simulink model "adaptiveCT"  (R2022a)
settings: Solver=VariableStepAuto  StartTime=0.0  StopTime=timeSpan  RelTol=1e-4
values from neighbouring files (symbols this model uses):
  B = [zeros(n);       eye(n)]    [adaptiveCT_main.m]
  K_p = 50 * eye(n)    [adaptiveCT_main.m]
  K_v = 10 * eye(n)    [adaptiveCT_main.m]
  max_tau = 100 * [1 1 1 1 1 1]    [adaptiveCT_main.m]
  P = lyap(A',Q)    [adaptiveCT_main.m]
  R = 10 * eye(n * 10)    [adaptiveCT_main.m]
undefined symbols (not defined in the file or in its folder): pi_est_0, pi_real
(part 2 of 5)

== matlab function adaptiveCT/Sistema/MATLAB Function1 ==
  data: q input; dq input; C_out output; parms input
function C_out = myCoriolis(q, dq, parms)

    % https://github.com/cdsousa/SymPyBotics

    %% Denavit-Hartenberg
    a2 = 0.4318;    a3 = 0.0203;
    d3 = 0.15005;   d4 = 0.4318;

    %% Variabili di giunto
    % q1 = q(1);  dq1 = dq(1);   ddq1 = ddq(1);
    % q2 = q(2);  dq2 = dq(2);   ddq2 = ddq(2);
    % q3 = q(3);  dq3 = dq(3);   ddq3 = ddq(3);
    % q4 = q(4);  dq4 = dq(4);   ddq4 = ddq(4);
    % q5 = q(5);  dq5 = dq(5);   ddq5 = ddq(5);
    % q6 = q(6);  dq6 = dq(6);   ddq6 = ddq(6);

    %% parms
    % (L_1xx, L_1xy, L_1xz, L_1yy, L_1yz, L_1zz, l_1x, l_1y, l_1z, m_1, L_2xx, L_2xy, L_2xz, L_2yy, L_2yz, L_2zz, l_2x, l_2y, l_2z, m_2, L_3xx, L_3xy, L_3xz, L_3yy, L_3yz, L_3zz, l_3x, l_3y, l_3z, m_3, L_4xx, L_4xy, L_4xz, L_4yy, L_4yz, L_4zz, l_4x, l_4y, l_4z, m_4, L_5xx, L_5xy, L_5xz, L_5yy, L_5yz, L_5zz, l_5x, l_5y, l_5z, m_5, L_6xx, L_6xy, L_6xz, L_6yy, L_6yz, L_6zz, l_6x, l_6y, l_6z, m_6)
    % Where:
    % L is the link inertia tensor computed about the link frame;
    % l is the link first moment of inertia;
    % m is the link mass.
    % These are the so-called barycentric parameters, with respect to which the dynamic model is linear.


    x0 = sin(q(2));
    x1 = cos(q(2));
    x2 = parms(13)*x0 + parms(15)*x1;
    x3 = ((x1)*(x1));
    x4 = -a2;
    x5 = ((x0)*(x0));
    x6 = x1*(x3*x4 + x4*x5);
    x7 = parms(19)*x6;
    x8 = x0*x7 + x1*x2;
    x9 = cos(q(3));
    x10 = x0*x9;
    x11 = sin(q(3));
    x12 = x1*x11;
    x13 = x10 + x12;
    x14 = parms(28)*x13;
    x15 = -d3;
    x16 = x12*x15;
    x17 = x10*x15 + x16;
    x18 = parms(30)*x17;
    x19 = x14 + x18;
    x20 = -x6;
    x21 = x1*x9;
    x22 = a3*((x11)*(x11)) + a3*((x9)*(x9));
    x23 = x0*x11;
    x24 = -x23;
    x25 = x20 + x21*x22 + x22*x24;
    x26 = -x17;
    x27 = x21 + x24;
    x28 = -x13;
    x29 = parms(27)*x27 + parms(29)*x28 + parms(30)*x25;
    x30 = x19*x25 + x26*x29;
    x31 = sin(q(4));
    x32 = x13*x31;
    x33 = -x32;
    x34 = d4*x33 + x25*x31;
    x35 = d3*x21;
    x36 = d3*x24 + x35;
    x37 = cos(q(4));
    x38 = x34 + x36*x37;
    x39 = -x38;
    x40 = parms(35)*x27;
    x41 = x13*x37;
    x42 = parms(33)*x41;
    x43 = parms(36)*x32 + parms(37)*x17 + x42;
    x44 = x40 + x43;
    x45 = parms(38)*x39 + x44;
    x46 = cos(q(5));
    x47 = x27*x46;
    x48 = sin(q(5));
    x49 = -x48;
    x50 = x41*x49;
    x51 = x47 + x50;
    x52 = parms(57)*x51;
    x53 = -x25;
    x54 = d4*x41 + x37*x53;
    x55 = x31*x36 + x54;
    x56 = -x55;
    x57 = cos(q(6));
    x58 = x17*x48;
    x59 = x38*x46 + x58;
    x60 = sin(q(6));
    x61 = -x60;
    x62 = x56*x57 + x59*x61;
    x63 = -parms(59);
    x64 = x27*x48;
    x65 = x41*x46;
    x66 = x64 + x65;
    x67 = x57*x66;
    x68 = x33*x60;
    x69 = x67 + x68;
    x70 = x63*x69;
    x71 = parms(60)*x62 + x52 + x70;
    x72 = x17*x46;
    x73 = x38*x49 + x72;
    x74 = -x73;
    x75 = x33*x57;
    x76 = x61*x66;
    x77 = x75 + x76;
    x78 = parms(53)*x69 + parms(55)*x77;
    x79 = parms(56)*x51;
    x80 = -parms(58);
    x81 = x56*x60 + x57*x59;
    x82 = parms(57)*x62 + x78 + x79 + x80*x81;
    x83 = -parms(57);
    x84 = parms(58)*x69 + x77*x83;
    x85 = parms(60)*x73 + x84;
    x86 = -x51;
    x87 = parms(52)*x69 + parms(54)*x77;
    x88 = parms(55)*x51;
    x89 = parms(59)*x81 + x73*x83 + x87 + x88;
    x90 = x62*x85 + x71*x74 + x77*x82 + x86*x89;
    x91 = parms(45)*x33;
    x92 = -x59;
    x93 = parms(43)*x66 + parms(46)*x51;
    x94 = parms(47)*x56 + parms(48)*x92 + x91 + x93;
    x95 = parms(48)*x66;
    x96 = -x33;
    x97 = parms(47)*x96;
    x98 = x95 + x97;
    x99 = parms(50)*x73 + x98;
    x100 = parms(53)*x51;
    x101 = parms(52)*x77;
    x102 = parms(51)*x69 + x101;
    x103 = parms(58)*x73 + x100 + x102 + x62*x63;
    x104 = parms(59)*x77;
    x105 = x51*x80;
    x106 = parms(60)*x81 + x104 + x105;
    x107 = -x69;
    x108 = x103*x51 + x106*x73 + x107*x82 - x81*x85;
    x109 = parms(44)*x33;
    x110 = parms(42)*x66 + parms(45)*x51;
    x111 = parms(47)*x74 + parms(49)*x59 + x109 + x110;
    x112 = -parms(49);
    x113 = parms(47)*x51 + x112*x66;
    x114 = parms(50)*x56 + x113;
    x115 = x108*x61 + x111*x86 + x114*x74 + x33*x94 + x56*x99 + x57*x90;
    x116 = parms(38)*x41;
    x117 = -x27;
    x118 = parms(37)*x117;
    x119 = x116 + x118;
    x120 = parms(40)*x55 + x119;
    x121 = -x77;
    x122 = x103*x121 - x106*x62 + x69*x89 + x71*x81;
    x123 = parms(42)*x33;
    x124 = parms(43)*x51;
    x125 = parms(41)*x66 + x124;
    x126 = parms(48)*x73 + x112*x56 + x123 + x125;
    x127 = parms(49)*x33;
    x128 = parms(48)*x86;
    x129 = x127 + x128;
    x130 = parms(50)*x59 + x129;
    x131 = x111*x66 + x114*x59 + x122 + x126*x96 - x130*x56;
    x132 = parms(34)*x27;
    x133 = parms(32)*x41 + parms(35)*x32;
    x134 = x132 + x133;
    x135 = parms(37)*x56 + parms(39)*x38 + x134;
    x136 = -parms(39);
    x137 = parms(37)*x32 + parms(40)*x17 + x136*x41;
    x138 = x115*x46 + x120*x17 + x131*x49 + x135*x33 + x137*x56 + x27*x45;
    x139 = -x66;
    x140 = -x108*x57 - x126*x51 - x130*x73 - x139*x94 - x60*x90 - x92*x99;
    x141 = parms(32)*x27;
    x142 = parms(31)*x41 + parms(33)*x32 + x136*x17;
    x143 = x141 + x142;
    x144 = parms(38)*x55 + x143;
    x145 = parms(39)*x27;
    x146 = parms(38)*x33;
    x147 = parms(40)*x38 + x145 + x146;
    x148 = x117*x144 + x135*x41 + x137*x38 + x140 + x147*x26;
    x149 = parms(22)*x13 + parms(25)*x27;
    x150 = parms(27)*x26 + x149;
    x151 = parms(29)*x36 + x150;
    x152 = x71*x86 + x77*x85;
    x153 = x106*x51 + x107*x85;
    x154 = x137*x41;
    x155 = x117*x147 - x130*x51 - x139*x99 - x152*x60 - x153*x57 + x154;
    x156 = d4*x37;
    x157 = x114*x86 + x152*x57 + x153*x61 + x33*x99;
    x158 = x106*x121 + x114*x66 + x130*x96 + x69*x71;
    x159 = x137*x33;
    x160 = x120*x27 + x157*x46 + x158*x49 + x159;
    x161 = d4*x31;
    x162 = x117*x151 + x138*x37 + x148*x31 + x155*x156 - x160*x161 + x30;
    x163 = -x41;
    x164 = x115*x48 + x120*x39 + x131*x46 + x144*x32 + x147*x55 + x163*x45;
    x165 = parms(28)*x117;
    x166 = parms(30)*x36 + x165;
    x167 = x13*x151 + x164 + x166*x53 + x29*x36;
    x168 = -x11;
    x169 = x117*x29;
    x170 = x155*x31 + x160*x37 + x169;
    x171 = x11*x15;
    x172 = x13*x29;
    x173 = x120*x163 + x147*x32 + x157*x48 + x158*x46 + x172;
    x174 = x173*x9;
    x175 = x19*x28;
    x176 = -x37;
    x177 = x155*x176 + x160*x31 + x166*x27 + x175;
    x178 = x177*x22;
    x179 = -x0;
    x180 = x1*x7 + x179*x2;
    x181 = -parms(19);
    x182 = x181*x3 + x181*x5;
    x183 = x0*(x15*x174 + x162*x9 + x167*x168 + x168*x178 + x170*x171 + x8) + x1*(d3*x170*x9 + x11*x162 + x167*x9 + x171*x173 + x178*x9 + x180) + x6*(-x177 + x182);
    x184 = -x1;
    x185 = parms(17)*x184 + parms(18)*x0 + parms(20)*x6;
    x186 = a2*x0;
    x187 = a2*parms(17) + parms(16) + x2;
    x188 = x11*x179 + x21;
    x189 = x179*x9;
    x190 = -x12;
    x191 = x189 + x190;
    x192 = x15*x23 + x35;
    x193 = a2*x11;
    x194 = x192 + x193;
    x195 = parms(28)*x194;
    x196 = x171*x179 - x35;
    x197 = x188*x37;
    x198 = x188*x31;
    x199 = d3*x189 + x16;
    x200 = -x186 + x189*x22 + x190*x22;
    x201 = x156*x188 + x176*x200 + x199*x31;
    x202 = a2*x9 + x22;
    x203 = x17 + x202;
    x204 = -x161;
    x205 = x204 + x54;
    x206 = x194*x31 + x205;
    x207 = -x31;
    x208 = x207 + x41;
    x209 = parms(38)*x208 + x118;
    x210 = parms(40)*x206 + x209;
    x211 = x191*x48 + x197*x46;
    x212 = -x198;
    x213 = x191*x46 + x197*x49;
    x214 = x188*x204 + x199*x37 + x200*x31;
    x215 = x196*x46 + x214*x49;
    x216 = x32 + x37;
    x217 = -x216;
    x218 = -x206;
    x219 = -parms(48);
    x220 = -x156;
    x221 = x220 + x34;
    x222 = x194*x37 + x221;
    x223 = x203*x48 + x222*x46;
    x224 = x208*x46 + x64;
    x225 = x208*x49 + x47;
    x226 = parms(43)*x224 + parms(45)*x217 + parms(46)*x225;
    x227 = parms(47)*x218 + x219*x223 + x226;
    x228 = x203*x46 + x222*x49;
    x229 = -parms(47);
    x230 = parms(48)*x224 + x217*x229;
    x231 = parms(50)*x228 + x230;
    x232 = x211*x57 + x212*x60;
    x233 = x211*x61 + x212*x57;
    x234 = x217*x57 + x224*x61;
    x235 = x218*x57 + x223*x61;
    x236 = x218*x60 + x223*x57;
    x237 = x217*x60 + x224*x57;
    x238 = parms(53)*x237 + parms(55)*x234 + parms(56)*x225;
    x239 = parms(57)*x235 + x236*x80 + x238;
    x240 = parms(58)*x237 + x234*x83;
    x241 = parms(60)*x228 + x240;
    x242 = -x201;
    x243 = x196*x48 + x214*x46;
    x244 = x242*x57 + x243*x61;
    x245 = parms(52)*x237 + parms(54)*x234 + parms(55)*x225;
    x246 = parms(59)*x236 + x228*x83 + x245;
    x247 = -x225;
    x248 = parms(57)*x225 + x237*x63;
    x249 = parms(60)*x235 + x248;
    x250 = -x228;
    x251 = parms(51)*x232 + parms(52)*x233 + parms(53)*x213 + parms(58)*x215 + x234*x239 + x235*x241 + x244*x63 + x246*x247 + x249*x250;
    x252 = parms(42)*x224 + parms(44)*x217 + parms(45)*x225;
    x253 = parms(49)*x223 + x228*x229 + x252;
    x254 = parms(47)*x225 + x112*x224;
    x255 = parms(50)*x218 + x254;
    x256 = x242*x60 + x243*x57;
    x257 = parms(51)*x237 + parms(52)*x234 + parms(53)*x225;
    x258 = parms(58)*x228 + x235*x63 + x257;
    x259 = parms(59)*x234 + x225*x80;
    x260 = parms(60)*x236 + x259;
    x261 = -x237;
    x262 = parms(52)*x232 + parms(54)*x233 + parms(55)*x213 + parms(59)*x256 + x215*x83 + x225*x258 + x228*x260 - x236*x241 + x239*x261;
    x263 = parms(41)*x211 + parms(42)*x212 + parms(43)*x213 + parms(48)*x215 + x112*x242 + x217*x227 + x218*x231 + x247*x253 + x250*x255 + x251*x57 + x262*x61;
    x264 = -x222;
    x265 = parms(33)*x208 + parms(36)*x216 + x40;
    x266 = parms(37)*x203 + parms(38)*x264 + x265;
    x267 = -parms(37);
    x268 = parms(32)*x208 + parms(35)*x216 + x132;
    x269 = parms(39)*x222 + x206*x267 + x268;
    x270 = parms(37)*x216 + x136*x208;
    x271 = parms(40)*x203 + x270;
    x272 = -x234;
    x273 = parms(53)*x232 + parms(55)*x233 + parms(56)*x213 + parms(57)*x244 - x235*x260 + x236*x249 + x237*x246 + x256*x80 + x258*x272;
    x274 = parms(41)*x224 + parms(42)*x217 + parms(43)*x225;
    x275 = parms(48)*x228 + x112*x218 + x274;
    x276 = -x217;
    x277 = parms(49)*x217 + x219*x225;
    x278 = parms(50)*x223 + x277;
    x279 = parms(43)*x211 + parms(45)*x212 + parms(46)*x213 + parms(47)*x242 - x218*x278 + x219*x243 + x223*x255 + x224*x253 + x273 + x275*x276;
    x280 = parms(31)*x197 + parms(32)*x191 + parms(33)*x198 + parms(38)*x201 + x136*x196 + x203*x210 + x217*x269 + x218*x271 + x263*x46 + x266*x27 + x279*x49;
    x281 = -x224;
    x282 = -parms(42)*x211 - parms(44)*x212 - parms(45)*x213 - parms(49)*x243 - x215*x229 + x223*x231 - x225*x275 - x227*x281 - x228*x278 - x251*x60 - x262*x57;
    x283 = -parms(38);
    x284 = parms(38)*x217 + x145;
    x285 = parms(40)*x222 + x284;
    x286 = -x203;
    x287 = parms(31)*x208 + parms(33)*x216 + x141;
    x288 = parms(38)*x206 + x136*x203 + x287;
    x289 = parms(33)*x197 + parms(35)*x191 + parms(36)*x198 + parms(37)*x196 + x117*x288 + x208*x269 + x214*x283 + x222*x271 + x282 + x285*x286;
    x290 = parms(30)*x203;
    x291 = parms(27) + x14;
    x292 = x290 + x291;
    x293 = -parms(29);
    x294 = -parms(27);
    x295 = -parms(24) + x149;
    x296 = parms(29)*x194 + x203*x294 + x295;
    x297 = parms(59)*x233 + parms(60)*x256 + x213*x80 + x234*x241 + x247*x249;
    x298 = parms(57)*x213 + parms(60)*x244 + x225*x260 + x232*x63 + x241*x261;
    x299 = parms(38)*x197 + parms(40)*x201 - parms(47)*x213 - parms(50)*x242 - x112*x211 + x117*x285 + x191*x267 + x208*x271 - x225*x278 - x231*x281 - x297*x60 - x298*x57;
    x300 = parms(49)*x212 + parms(50)*x243 + x213*x219 + x217*x231 + x247*x255 + x297*x57 + x298*x61;
    x301 = parms(48)*x211 + parms(50)*x215 + parms(58)*x232 + parms(60)*x215 + x212*x229 + x224*x255 + x233*x83 + x237*x249 + x260*x272 + x276*x278;
    x302 = parms(38)*x212 + parms(39)*x191 + parms(40)*x214 + x210*x27 + x217*x271 + x300*x46 + x301*x49;
    x303 = parms(23)*x13;
    x304 = parms(25) + parms(26)*x117 + parms(27)*x53 - x303;
    x305 = parms(21)*x188 + parms(23)*x191 + parms(28)*x196 + x117*x296 + x156*x299 + x195 + x200*x293 + x204*x302 + x25*x292 + x280*x37 + x286*x29 + x289*x31 + x304;
    x306 = parms(12)*x0;
    x307 = parms(14)*x1;
    x308 = -x208;
    x309 = parms(32)*x197 + parms(34)*x191 + parms(35)*x198 + parms(39)*x214 + x201*x267 + x206*x285 + x210*x264 + x216*x288 + x263*x48 + x266*x308 + x279*x46;
    x310 = parms(21)*x13 + parms(29)*x53;
    x311 = parms(23)*x27;
    x312 = x310 + x311;
    x313 = -parms(22);
    x314 = x312 + x313;
    x315 = parms(28)*x203 + x314;
    x316 = -parms(28);
    x317 = x165 + x293;
    x318 = parms(30)*x194 + x317;
    x319 = parms(23)*x188 + parms(26)*x191 + parms(27)*x200 + x13*x296 + x194*x29 + x199*x316 + x309 + x315 + x318*x53;
    x320 = a2*parms(20) + parms(17) + parms(19)*x179;
    x321 = -x14 + x169 + x294;
    x322 = parms(30)*x199 + x191*x316 - x290 + x299*x31 + x302*x37 + x321;
    x323 = parms(28)*x188 + parms(30)*x196 + parms(37)*x198 + parms(40)*x196 + x136*x197 + x172 + x210*x308 + x216*x285 + x300*x48 + x301*x46 + x318;
    x324 = x323*x9;
    x325 = parms(27)*x191 + parms(30)*x200 + x176*x299 + x188*x293 + x27*x318 + x28*x292 + x302*x31;
    x326 = x22*x325;
    x327 = -parms(15);
    x328 = -parms(18);
    x329 = parms(19)*x1 + x328;
    x330 = -parms(17);
    x331 = parms(12)*x1;
    x332 = parms(11)*x0 + parms(18)*x6;
    x333 = parms(13) + parms(19)*x4;
    x334 = -x183;
    x335 = parms(28)*x193;
    x336 = parms(25) + x335;
    x337 = parms(38)*x207;
    x338 = x193*x31;
    x339 = x204 + x338;
    x340 = parms(40)*x339;
    x341 = x337 + x340;
    x342 = x193*x37;
    x343 = x220 + x342;
    x344 = -x339;
    x345 = parms(32)*x207 + parms(35)*x37;
    x346 = parms(37)*x344 + parms(39)*x343 + x345;
    x347 = parms(37)*x37 + x136*x207;
    x348 = parms(40)*x202 + x347;
    x349 = x344*x348;
    x350 = x176*x346 + x202*x341 + x349;
    x351 = x202*x48 + x343*x46;
    x352 = -x351;
    x353 = parms(48)*x352;
    x354 = parms(47)*x344 + x353;
    x355 = x207*x46;
    x356 = x207*x49;
    x357 = parms(43)*x355 + parms(46)*x356;
    x358 = parms(45)*x176;
    x359 = x357 + x358;
    x360 = x354 + x359;
    x361 = x202*x46 + x343*x49;
    x362 = parms(50)*x361;
    x363 = parms(48)*x355;
    x364 = -x176;
    x365 = parms(47)*x364;
    x366 = x363 + x365;
    x367 = x362 + x366;
    x368 = -x356;
    x369 = -x361;
    x370 = parms(47)*x369 + parms(49)*x351;
    x371 = parms(42)*x355 + parms(45)*x356;
    x372 = parms(44)*x176;
    x373 = x371 + x372;
    x374 = x370 + x373;
    x375 = parms(50)*x344;
    x376 = parms(47)*x356 + x112*x355;
    x377 = x375 + x376;
    x378 = x369*x377;
    x379 = x176*x360 + x344*x367 + x368*x374 + x378;
    x380 = x176*x57;
    x381 = x355*x61;
    x382 = x380 + x381;
    x383 = x344*x57 + x351*x61;
    x384 = x344*x60 + x351*x57;
    x385 = parms(57)*x383 + x384*x80;
    x386 = x176*x60;
    x387 = x355*x57;
    x388 = x386 + x387;
    x389 = parms(53)*x388 + parms(55)*x382;
    x390 = parms(56)*x356;
    x391 = x389 + x390;
    x392 = x385 + x391;
    x393 = parms(60)*x361;
    x394 = parms(58)*x388 + x382*x83;
    x395 = x393 + x394;
    x396 = x383*x395;
    x397 = parms(59)*x384 + x361*x83;
    x398 = parms(52)*x388 + parms(54)*x382;
    x399 = parms(55)*x356;
    x400 = x398 + x399;
    x401 = x397 + x400;
    x402 = parms(60)*x383;
    x403 = parms(57)*x356;
    x404 = x388*x63;
    x405 = x403 + x404;
    x406 = x402 + x405;
    x407 = x368*x401 + x369*x406 + x382*x392 + x396;
    x408 = parms(58)*x361 + x383*x63;
    x409 = parms(52)*x382;
    x410 = parms(51)*x388 + x409;
    x411 = parms(53)*x356;
    x412 = x410 + x411;
    x413 = x408 + x412;
    x414 = parms(60)*x384;
    x415 = parms(59)*x382;
    x416 = x356*x80;
    x417 = x415 + x416;
    x418 = x414 + x417;
    x419 = -x388;
    x420 = -x384;
    x421 = x395*x420;
    x422 = x356*x413 + x361*x418 + x392*x419 + x421;
    x423 = x379 + x407*x57 + x422*x61;
    x424 = x351*x377;
    x425 = parms(48)*x361 + x112*x344;
    x426 = parms(43)*x356;
    x427 = parms(41)*x355 + x426;
    x428 = parms(42)*x176;
    x429 = x427 + x428;
    x430 = x425 + x429;
    x431 = -x344;
    x432 = parms(50)*x351;
    x433 = parms(49)*x176;
    x434 = parms(48)*x368;
    x435 = x433 + x434;
    x436 = x432 + x435;
    x437 = x355*x374 + x364*x430 + x424 + x431*x436;
    x438 = -x382;
    x439 = -x383;
    x440 = x384*x406 + x388*x401 + x413*x438 + x418*x439;
    x441 = x437 + x440;
    x442 = x350 + x423*x46 + x441*x49;
    x443 = x343*x348;
    x444 = -x202;
    x445 = parms(38)*x176;
    x446 = parms(40)*x343 + x445;
    x447 = x207*x346 + x443 + x444*x446;
    x448 = -x355;
    x449 = x352*x367 + x356*x430 + x360*x448 + x361*x436;
    x450 = -x407*x60 - x422*x57 - x449;
    x451 = x447 + x450;
    x452 = x356*x436 + x367*x448;
    x453 = x382*x395;
    x454 = x368*x406 + x453;
    x455 = x395*x419;
    x456 = x356*x418 + x455;
    x457 = x207*x348;
    x458 = -x452 - x454*x60 - x456*x57 + x457;
    x459 = x368*x377;
    x460 = x176*x367 + x459;
    x461 = x454*x57 + x456*x61 + x460;
    x462 = x176*x348;
    x463 = x355*x377;
    x464 = x364*x436 + x463;
    x465 = x388*x406 + x418*x438 + x464;
    x466 = x46*x461 + x462 + x465*x49;
    x467 = x156*x458 + x204*x466 + x31*x451 + x336 + x37*x442;
    x468 = parms(28)*x202 + x313;
    x469 = parms(31)*x207;
    x470 = parms(33)*x37 + x469;
    x471 = parms(38)*x339 + x136*x202 + x470;
    x472 = parms(37)*x202;
    x473 = -x343;
    x474 = parms(33)*x207;
    x475 = parms(36)*x37;
    x476 = x474 + x475;
    x477 = parms(38)*x473 + x472 + x476;
    x478 = -x207;
    x479 = x339*x446 + x341*x473 + x37*x471 + x477*x478;
    x480 = x423*x48 + x441*x46 + x479;
    x481 = x468 + x480;
    x482 = parms(30)*x202;
    x483 = x294 - x482;
    x484 = x31*x458 + x37*x466 + x483;
    x485 = x341*x478 + x37*x446;
    x486 = parms(30)*x193;
    x487 = x293 + x486;
    x488 = x46*x465 + x461*x48 + x485 + x487;
    x489 = x488*x9;
    x490 = x176*x458 + x31*x466;
    x491 = x22*x490;
    x492 = x0*(x15*x489 + x168*x481 + x168*x491 + x171*x484 + x327 + x467*x9) + x1*(d3*x484*x9 + x11*x467 + x171*x488 + x333 + x481*x9 + x491*x9) - x490*x6;
    x493 = -x492;
    x494 = -x192;
    x495 = x27*x37;
    x496 = x27*x31;
    x497 = a3*x28;
    x498 = x156*x27 + x17*x31 + x176*x497;
    x499 = a3 + x17;
    x500 = x192*x37;
    x501 = x221 + x500;
    x502 = parms(37)*x499 + x265 + x283*x501;
    x503 = x192*x31;
    x504 = x205 + x503;
    x505 = parms(40)*x504 + x209;
    x506 = x28*x48 + x46*x495;
    x507 = -x496;
    x508 = x28*x46 + x49*x495;
    x509 = x117*x161 + x17*x37 + x31*x497;
    x510 = x46*x494 + x49*x509;
    x511 = -x504;
    x512 = x46*x501 + x48*x499;
    x513 = parms(47)*x511 + x219*x512 + x226;
    x514 = x46*x499 + x49*x501;
    x515 = parms(50)*x514 + x230;
    x516 = x506*x57 + x507*x60;
    x517 = x506*x61 + x507*x57;
    x518 = x511*x57 + x512*x61;
    x519 = x511*x60 + x512*x57;
    x520 = parms(57)*x518 + x238 + x519*x80;
    x521 = parms(60)*x514 + x240;
    x522 = -x498;
    x523 = x46*x509 + x48*x494;
    x524 = x522*x57 + x523*x61;
    x525 = parms(59)*x519 + x245 + x514*x83;
    x526 = parms(60)*x518 + x248;
    x527 = -x514;
    x528 = parms(51)*x516 + parms(52)*x517 + parms(53)*x508 + parms(58)*x510 + x234*x520 + x247*x525 + x518*x521 + x524*x63 + x526*x527;
    x529 = parms(49)*x512 + x229*x514 + x252;
    x530 = parms(50)*x511 + x254;
    x531 = x522*x60 + x523*x57;
    x532 = parms(58)*x514 + x257 + x518*x63;
    x533 = parms(60)*x519 + x259;
    x534 = parms(52)*x516 + parms(54)*x517 + parms(55)*x508 + parms(59)*x531 + x225*x532 + x261*x520 + x510*x83 + x514*x533 - x519*x521;
    x535 = parms(41)*x506 + parms(42)*x507 + parms(43)*x508 + parms(48)*x510 + x112*x522 + x217*x513 + x247*x529 + x511*x515 + x527*x530 + x528*x57 + x534*x61;
    x536 = parms(39)*x501 + x267*x504 + x268;
    x537 = parms(40)*x499 + x270;
    x538 = parms(53)*x516 + parms(55)*x517 + parms(56)*x508 + parms(57)*x524 + x237*x525 + x272*x532 - x518*x533 + x519*x526 + x531*x80;
    x539 = parms(48)*x514 + x112*x511 + x274;
    x540 = parms(50)*x512 + x277;
    x541 = parms(43)*x506 + parms(45)*x507 + parms(46)*x508 + parms(47)*x522 + x219*x523 + x224*x529 + x276*x539 - x511*x540 + x512*x530 + x538;
    x542 = parms(31)*x495 + parms(32)*x28 + parms(33)*x496 + parms(38)*x498 + x136*x494 + x217*x536 + x27*x502 + x46*x535 + x49*x541 + x499*x505 + x511*x537;
    x543 = -parms(42)*x506 - parms(44)*x507 - parms(45)*x508 - parms(49)*x523 - x225*x539 - x229*x510 - x281*x513 + x512*x515 - x514*x540 - x528*x60 - x534*x57;
    x544 = parms(38)*x504 + x136*x499 + x287;
    x545 = parms(40)*x501 + x284;
    x546 = -x499;
    x547 = parms(33)*x495 + parms(35)*x28 + parms(36)*x496 + parms(37)*x494 + x117*x544 + x208*x536 + x283*x509 + x501*x537 + x543 + x545*x546;
    x548 = parms(30)*x499;
    x549 = x291 + x548;
    x550 = parms(29)*x192;
    x551 = x294*x499 + x295 + x550;
    x552 = parms(59)*x517 + parms(60)*x531 + x234*x521 + x247*x526 + x508*x80;
    x553 = parms(57)*x508 + parms(60)*x524 + x225*x533 + x261*x521 + x516*x63;
    x554 = parms(38)*x495 + parms(40)*x498 - parms(47)*x508 - parms(50)*x522 - x112*x506 + x117*x545 + x208*x537 - x225*x540 + x267*x28 - x281*x515 - x552*x60 - x553*x57;
    x555 = parms(49)*x507 + parms(50)*x523 + x217*x515 + x219*x508 + x247*x530 + x552*x57 + x553*x61;
    x556 = parms(48)*x506 + parms(50)*x510 + parms(58)*x516 + parms(60)*x510 + x224*x530 + x229*x507 + x237*x526 + x272*x533 + x276*x540 + x517*x83;
    x557 = parms(38)*x507 + parms(39)*x28 + parms(40)*x509 + x217*x537 + x27*x505 + x46*x555 + x49*x556;
    x558 = parms(21)*x27 + parms(23)*x28 + parms(28)*x192 + parms(28)*x494 + x117*x551 + x156*x554 + x204*x557 + x25*x549 + x29*x546 + x293*x497 + x304 + x31*x547 + x37*x542;
    x559 = parms(32)*x495 + parms(34)*x28 + parms(35)*x496 + parms(39)*x509 + x216*x544 + x267*x498 + x308*x502 + x46*x541 + x48*x535 - x501*x505 + x504*x545;
    x560 = parms(28)*x499;
    x561 = x192*x29;
    x562 = parms(30)*x192;
    x563 = x317 + x562;
    x564 = parms(26)*x28 + parms(27)*x497 + parms(28)*x26 + x13*x551 + x310 + 2*x311 + x313 + x53*x563 + x559 + x560 + x561;
    x565 = x18 + x28*x316 + x31*x554 + x321 + x37*x557 - x548;
    x566 = parms(30)*x494 + parms(37)*x496 + parms(40)*x494 + x136*x495 + x172 + x216*x545 + x293 + x308*x505 + x46*x556 + x48*x555 + x562;
    x567 = x566*x9;
    x568 = parms(27)*x28 + parms(29)*x117 + parms(30)*x497 + x176*x554 + x27*x563 + x28*x549 + x31*x557;
    x569 = x22*x568;
    x570 = parms(40)*x204;
    x571 = x337 + x570;
    x572 = -x204;
    x573 = parms(37)*x572 + parms(39)*x220 + x345;
    x574 = a3*parms(40) + x347;
    x575 = x572*x574;
    x576 = a3*x571 + x176*x573 + x575;
    x577 = a3*x48 + x220*x46;
    x578 = -x577;
    x579 = parms(48)*x578;
    x580 = parms(47)*x572 + x579;
    x581 = x359 + x580;
    x582 = a3*x46 + x220*x49;
    x583 = parms(50)*x582;
    x584 = x366 + x583;
    x585 = -x582;
    x586 = parms(47)*x585 + parms(49)*x577;
    x587 = x373 + x586;
    x588 = parms(50)*x572;
    x589 = x376 + x588;
    x590 = x585*x589;
    x591 = x176*x581 + x368*x587 + x572*x584 + x590;
    x592 = x57*x572 + x577*x61;
    x593 = x57*x577 + x572*x60;
    x594 = parms(57)*x592 + x593*x80;
    x595 = x391 + x594;
    x596 = parms(60)*x582;
    x597 = x394 + x596;
    x598 = x592*x597;
    x599 = parms(59)*x593 + x582*x83;
    x600 = x400 + x599;
    x601 = parms(60)*x592;
    x602 = x405 + x601;
    x603 = x368*x600 + x382*x595 + x585*x602 + x598;
    x604 = parms(58)*x582 + x592*x63;
    x605 = x412 + x604;
    x606 = parms(60)*x593;
    x607 = x417 + x606;
    x608 = -x593;
    x609 = x597*x608;
    x610 = x356*x605 + x419*x595 + x582*x607 + x609;
    x611 = x57*x603 + x591 + x61*x610;
    x612 = x577*x589;
    x613 = parms(48)*x582 + x112*x572;
    x614 = x429 + x613;
    x615 = -x572;
    x616 = parms(50)*x577;
    x617 = x435 + x616;
    x618 = x355*x587 + x364*x614 + x612 + x615*x617;
    x619 = -x592;
    x620 = x388*x600 + x438*x605 + x593*x602 + x607*x619;
    x621 = x618 + x620;
    x622 = x46*x611 + x49*x621 + x576;
    x623 = x220*x574;
    x624 = parms(40)*x220 + x445;
    x625 = -a3;
    x626 = x207*x573 + x623 + x624*x625;
    x627 = x356*x614 + x448*x581 + x578*x584 + x582*x617;
    x628 = -x57*x610 - x60*x603 - x627;
    x629 = x626 + x628;
    x630 = x356*x617 + x448*x584;
    x631 = x382*x597;
    x632 = x368*x602 + x631;
    x633 = x419*x597;
    x634 = x356*x607 + x633;
    x635 = x207*x574;
    x636 = -x57*x634 - x60*x632 - x630 + x635;
    x637 = x368*x589;
    x638 = x176*x584 + x637;
    x639 = x57*x632 + x61*x634 + x638;
    x640 = x176*x574;
    x641 = x355*x589;
    x642 = x364*x617 + x641;
    x643 = x388*x602 + x438*x607 + x642;
    x644 = x46*x639 + x49*x643 + x640;
    x645 = parms(25) + x156*x636 + x204*x644 + x31*x629 + x37*x622;
    x646 = a3*parms(28) + x313;
    x647 = a3*x136 + parms(38)*x204 + x470;
    x648 = a3*parms(37);
    x649 = -x220;
    x650 = parms(38)*x649 + x476 + x648;
    x651 = x204*x624 + x37*x647 + x478*x650 + x571*x649;
    x652 = x46*x621 + x48*x611 + x651;
    x653 = x646 + x652;
    x654 = parms(30)*x625 + x294;
    x655 = x31*x636 + x37*x644 + x654;
    x656 = x37*x624 + x478*x571;
    x657 = x293 + x46*x643 + x48*x639 + x656;
    x658 = x657*x9;
    x659 = x176*x636 + x31*x644;
    x660 = x22*x659;
    x661 = x0*(x15*x658 + x168*x653 + x168*x660 + x171*x655 + x645*x9) + x1*(d3*x655*x9 + x11*x645 + x171*x657 + x653*x9 + x660*x9) - x6*x659;
    x662 = -x661;
    x663 = -x193;
    x664 = x202 + x625;
    x665 = x31*x664;
    x666 = a3 + x202;
    x667 = -2*x31;
    x668 = -2*x161 + x338;
    x669 = parms(38)*x667 + parms(40)*x668;
    x670 = x37*x664;
    x671 = x46*x663 + x49*x670;
    x672 = 2*x37;
    x673 = -x672;
    x674 = x46*x667;
    x675 = x49*x667;
    x676 = -x668;
    x677 = -2*x156 + x342;
    x678 = x46*x677 + x48*x666;
    x679 = parms(43)*x674 + parms(45)*x673 + parms(46)*x675 + parms(47)*x676 + x219*x678;
    x680 = x46*x666 + x49*x677;
    x681 = parms(48)*x674 + parms(50)*x680 + x229*x673;
    x682 = x57*x673 + x61*x674;
    x683 = x57*x674 + x60*x673;
    x684 = x57*x676 + x61*x678;
    x685 = x57*x678 + x60*x676;
    x686 = parms(53)*x683 + parms(55)*x682 + parms(56)*x675 + parms(57)*x684 + x685*x80;
    x687 = parms(58)*x683 + parms(60)*x680 + x682*x83;
    x688 = -x665;
    x689 = x46*x670 + x48*x663;
    x690 = x57*x688 + x61*x689;
    x691 = parms(52)*x683 + parms(54)*x682 + parms(55)*x675 + parms(59)*x685 + x680*x83;
    x692 = -x675;
    x693 = parms(57)*x675 + parms(60)*x684 + x63*x683;
    x694 = -x680;
    x695 = parms(58)*x671 + x63*x690 + x682*x686 + x684*x687 + x691*x692 + x693*x694;
    x696 = parms(42)*x674 + parms(44)*x673 + parms(45)*x675 + parms(49)*x678 + x229*x680;
    x697 = parms(47)*x675 + parms(50)*x676 + x112*x674;
    x698 = x57*x689 + x60*x688;
    x699 = parms(51)*x683 + parms(52)*x682 + parms(53)*x675 + parms(58)*x680 + x63*x684;
    x700 = parms(59)*x682 + parms(60)*x685 + x675*x80;
    x701 = -x683;
    x702 = parms(59)*x698 + x671*x83 + x675*x699 + x680*x700 - x685*x687 + x686*x701;
    x703 = parms(48)*x671 + x112*x688 + x57*x695 + x61*x702 + x673*x679 + x676*x681 + x692*x696 + x694*x697;
    x704 = parms(32)*x667 + parms(35)*x672 + parms(39)*x677 + x267*x668;
    x705 = parms(37)*x672 + parms(40)*x666 + x136*x667;
    x706 = -x682;
    x707 = parms(57)*x690 + x683*x691 - x684*x700 + x685*x693 + x698*x80 + x699*x706;
    x708 = parms(41)*x674 + parms(42)*x673 + parms(43)*x675 + parms(48)*x680 + x112*x676;
    x709 = -x673;
    x710 = parms(49)*x673 + parms(50)*x678 + x219*x675;
    x711 = parms(47)*x688 + x219*x689 + x674*x696 - x676*x710 + x678*x697 + x707 + x708*x709;
    x712 = parms(38)*x665 + x136*x663 + x46*x703 + x49*x711 + x666*x669 + x673*x704 + x676*x705;
    x713 = -x674;
    x714 = -parms(49)*x689 - x229*x671 - x57*x702 - x60*x695 - x675*x708 + x678*x681 - x679*x713 - x680*x710;
    x715 = parms(40)*x677 + x283*x672;
    x716 = parms(37)*x663 + x283*x670 - x666*x715 + x667*x704 + x677*x705 + x714;
    x717 = parms(60)*x698 + x682*x687 + x692*x693;
    x718 = parms(60)*x690 + x675*x700 + x687*x701;
    x719 = parms(40)*x665 - parms(50)*x688 - x57*x718 - x60*x717 + x667*x705 - x675*x710 - x681*x713;
    x720 = parms(50)*x689 + x57*x717 + x61*x718 + x673*x681 + x692*x697;
    x721 = parms(50)*x671 + parms(60)*x671 + x674*x697 + x683*x693 + x700*x706 + x709*x710;
    x722 = parms(40)*x670 + x46*x720 + x49*x721 + x673*x705;
    x723 = 4*parms(25) + parms(28)*x663 + x156*x719 + x204*x722 + x31*x716 + 2*x335 + x37*x712;
    x724 = -x667;
    x725 = parms(39)*x670 + x267*x665 + x46*x711 + x48*x703 + x668*x715 - x669*x677 + x672*(parms(31)*x667 + parms(33)*x672 + parms(38)*x668 + x136*x666) + x724*(parms(33)*x667 + parms(36)*x672 + parms(37)*x666 + x283*x677);
    x726 = -4*parms(22) + 2*parms(28)*x666 + x316*x664 + x725;
    x727 = parms(30)*x666;
    x728 = -4*parms(27) + parms(30)*x664 + x31*x719 + x37*x722 - 2*x727;
    x729 = -4*parms(29) + parms(30)*x663 + parms(40)*x663 + x46*x721 + x48*x720 + 2*x486 + x669*x724 + x672*x715;
    x730 = x729*x9;
    x731 = x176*x719 + x31*x722;
    x732 = x22*x731;
    x733 = x34 + x500;
    x734 = x27 + 1;
    x735 = x283*x733;
    x736 = x43 + x735;
    x737 = parms(35)*x734 + x736;
    x738 = x33*x46;
    x739 = x33*x49;
    x740 = x503 + x54;
    x741 = -x740;
    x742 = x49*x741;
    x743 = x48*x734 + x65;
    x744 = x49*x733 + x72;
    x745 = parms(50)*x744;
    x746 = parms(48)*x743 + x745 + x97;
    x747 = x163*x60 + x57*x738;
    x748 = x163*x57 + x61*x738;
    x749 = x61*x743 + x75;
    x750 = x57*x743 + x68;
    x751 = x46*x734 + x50;
    x752 = x46*x733 + x58;
    x753 = x57*x741 + x61*x752;
    x754 = x57*x752 + x60*x741;
    x755 = parms(57)*x753 + x754*x80;
    x756 = parms(53)*x750 + parms(55)*x749 + parms(56)*x751 + x755;
    x757 = parms(60)*x744;
    x758 = parms(58)*x750 + x749*x83 + x757;
    x759 = -x733;
    x760 = x46*x741;
    x761 = x57*x759 + x61*x760;
    x762 = parms(59)*x754 + x744*x83;
    x763 = parms(52)*x750 + parms(54)*x749 + parms(55)*x751 + x762;
    x764 = -x751;
    x765 = parms(60)*x753;
    x766 = parms(57)*x751 + x63*x750 + x765;
    x767 = -x744;
    x768 = parms(51)*x747 + parms(52)*x748 + parms(53)*x739 + parms(58)*x742 + x63*x761 + x749*x756 + x753*x758 + x763*x764 + x766*x767;
    x769 = parms(47)*x741 + x219*x752;
    x770 = parms(43)*x743 + parms(46)*x751 + x769 + x91;
    x771 = parms(49)*x752 + x229*x744;
    x772 = parms(42)*x743 + parms(45)*x751 + x109 + x771;
    x773 = parms(50)*x741;
    x774 = parms(47)*x751 + x112*x743 + x773;
    x775 = x57*x760 + x60*x759;
    x776 = parms(58)*x744 + x63*x753;
    x777 = parms(51)*x750 + parms(52)*x749 + parms(53)*x751 + x776;
    x778 = parms(60)*x754;
    x779 = parms(59)*x749 + x751*x80 + x778;
    x780 = -x750;
    x781 = -x754;
    x782 = parms(52)*x747 + parms(54)*x748 + parms(55)*x739 + parms(59)*x775 + x742*x83 + x744*x779 + x751*x777 + x756*x780 + x758*x781;
    x783 = parms(41)*x738 + parms(42)*x163 + parms(43)*x739 + parms(48)*x742 + x112*x759 + x33*x770 + x57*x768 + x61*x782 + x741*x746 + x764*x772 + x767*x774;
    x784 = parms(40)*x740;
    x785 = x116 + x267*x734 + x784;
    x786 = x137*x741;
    x787 = -x749;
    x788 = -x753;
    x789 = parms(53)*x747 + parms(55)*x748 + parms(56)*x739 + parms(57)*x761 + x750*x763 + x754*x766 + x775*x80 + x777*x787 + x779*x788;
    x790 = parms(50)*x752;
    x791 = x127 + x219*x751 + x790;
    x792 = -x741;
    x793 = parms(48)*x744 + x112*x741;
    x794 = parms(41)*x743 + parms(43)*x751 + x123 + x793;
    x795 = parms(43)*x738 + parms(45)*x163 + parms(46)*x739 + parms(47)*x759 + x219*x760 + x743*x772 + x752*x774 + x789 + x791*x792 + x794*x96;
    x796 = parms(39)*x733 + x267*x740;
    x797 = parms(34)*x734 + x133 + x796;
    x798 = parms(31)*x33 + parms(38)*x733 + x17*x785 + x33*x797 + x42 + x46*x783 + x49*x795 + x734*x737 + x786;
    x799 = -x743;
    x800 = -x752;
    x801 = -parms(42)*x738 - parms(44)*x163 - parms(45)*x739 - parms(49)*x760 - x229*x742 - x57*x782 - x60*x768 - x744*x791 - x746*x800 - x751*x794 - x770*x799;
    x802 = x137*x733;
    x803 = parms(38)*x740;
    x804 = x142 + x803;
    x805 = parms(32)*x734 + x804;
    x806 = -x734;
    x807 = parms(40)*x733 + x146;
    x808 = parms(39)*x734 + x807;
    x809 = parms(33)*x33 + parms(36)*x41 + x26*x808 + x283*x741 + x41*x797 + x801 + x802 + x805*x806;
    x810 = parms(59)*x748 + parms(60)*x775 + x739*x80 + x749*x758 + x764*x766;
    x811 = parms(57)*x739 + parms(60)*x761 + x63*x747 + x751*x779 + x758*x780;
    x812 = -parms(47)*x739 - parms(50)*x759 - x112*x738 + x154 - x57*x811 - x60*x810 - x746*x799 - x751*x791 + x806*x808 + x807;
    x813 = parms(49)*x163 + parms(50)*x760 + x219*x739 + x33*x746 + x57*x810 + x61*x811 + x764*x774;
    x814 = parms(48)*x738 + parms(50)*x742 + parms(58)*x747 + parms(60)*x742 + x163*x229 + x743*x774 + x748*x83 + x750*x766 + x779*x787 + x791*x96;
    x815 = parms(40)*x741 - x116 + x159 + x46*x813 + x49*x814 + x734*x785;
    x816 = x150 + x550;
    x817 = x117*x816 + x30;
    x818 = x156*x812 + x204*x815 + x31*x809 + x37*x798 + x817;
    x819 = parms(32)*x33 + parms(35)*x41 + parms(39)*x741 + x163*x737 + x267*x733 + x32*x805 + x46*x795 + x48*x783 + x740*x808 + x759*x785;
    x820 = x165 + x562;
    x821 = x13*x816 + x53*x820 + x561;
    x822 = x819 + x821;
    x823 = x169 + x31*x812 + x37*x815;
    x824 = parms(37)*x41 + parms(39)*x96 + x163*x785 + x172 + x32*x808 + x46*x814 + x48*x813;
    x825 = x824*x9;
    x826 = x175 + x27*x820;
    x827 = x176*x812 + x31*x815 + x826;
    x828 = x22*x827;
    x829 = x49*x60;
    x830 = x48*x57;
    x831 = parms(53)*x830 + parms(55)*x829;
    x832 = parms(56)*x46;
    x833 = x831 + x832;
    x834 = parms(52)*x830 + parms(54)*x829;
    x835 = parms(55)*x46;
    x836 = x834 + x835;
    x837 = -x46;
    x838 = x829*x833 + x836*x837;
    x839 = parms(42)*x48 + parms(45)*x46;
    x840 = x837*x839;
    x841 = parms(52)*x829;
    x842 = parms(51)*x830 + x841;
    x843 = parms(53)*x46;
    x844 = x842 + x843;
    x845 = -x830;
    x846 = x46*x844 + x833*x845;
    x847 = x57*x838 + x61*x846 + x840;
    x848 = x48*x839;
    x849 = -x829;
    x850 = x830*x836 + x844*x849;
    x851 = x848 + x850;
    x852 = parms(35) + x46*x847 + x49*x851;
    x853 = parms(43)*x48 + parms(46)*x46;
    x854 = parms(41)*x48;
    x855 = parms(43)*x46;
    x856 = x854 + x855;
    x857 = x46*x856 + x49*x853;
    x858 = -x57*x846 - x60*x838 - x857;
    x859 = -parms(32);
    x860 = x858 + x859;
    x861 = parms(58)*x830 + x829*x83;
    x862 = x829*x861;
    x863 = parms(57)*x46;
    x864 = x63*x830;
    x865 = x863 + x864;
    x866 = x837*x865 + x862;
    x867 = parms(59)*x829;
    x868 = x46*x80;
    x869 = x867 + x868;
    x870 = x845*x861;
    x871 = x46*x869 + x870;
    x872 = x219*((x46)*(x46)) + x219*((x48)*(x48));
    x873 = x136 - x57*x871 - x60*x866 - x872;
    x874 = parms(47)*x46 + parms(49)*x49;
    x875 = x837*x874;
    x876 = x57*x866 + x61*x871 + x875;
    x877 = x48*x874;
    x878 = x830*x865 + x849*x869 + x877;
    x879 = x267 + x46*x876 + x49*x878;
    x880 = x156*x873 + x204*x879 + x31*x860 + x37*x852;
    x881 = x46*x851 + x48*x847;
    x882 = x46*x878 + x48*x876;
    x883 = x882*x9;
    x884 = x31*x873 + x37*x879;
    x885 = x176*x873 + x31*x879;
    x886 = x22*x885;
    x887 = x0*(x15*x883 + x168*x881 + x168*x886 + x171*x884 + x880*x9) + x1*(d3*x884*x9 + x11*x880 + x171*x882 + x881*x9 + x886*x9) - x6*x885;
    x888 = -x887;
    x889 = x344*x49;
    x890 = x355 + x48;
    x891 = x356 + x46;
    x892 = parms(43)*x890 + parms(46)*x891 + x358;
    x893 = x354 + x892;
    x894 = x380 + x61*x890;
    x895 = x386 + x57*x890;
    x896 = parms(53)*x895 + parms(55)*x894 + parms(56)*x891;
    x897 = x385 + x896;
    x898 = parms(58)*x895 + x83*x894;
    x899 = x393 + x898;
    x900 = x344*x46;
    x901 = x473*x57 + x61*x900;
    x902 = parms(52)*x895 + parms(54)*x894 + parms(55)*x891;
    x903 = x397 + x902;
    x904 = -x891;
    x905 = parms(57)*x891 + x63*x895;
    x906 = x402 + x905;
    x907 = x176*x46;
    x908 = x478*x60 + x57*x907;
    x909 = x478*x57 + x61*x907;
    x910 = x176*x49;
    x911 = parms(51)*x908 + parms(52)*x909 + parms(53)*x910;
    x912 = parms(58)*x889 + x369*x906 + x383*x899 + x63*x901 + x894*x897 + x903*x904 + x911;
    x913 = parms(48)*x890 + x365;
    x914 = x362 + x913;
    x915 = parms(42)*x890 + parms(45)*x891 + x372;
    x916 = x370 + x915;
    x917 = x473*x60 + x57*x900;
    x918 = parms(51)*x895 + parms(52)*x894 + parms(53)*x891;
    x919 = x408 + x918;
    x920 = parms(59)*x894 + x80*x891;
    x921 = x414 + x920;
    x922 = -x895;
    x923 = parms(52)*x908 + parms(54)*x909 + parms(55)*x910;
    x924 = parms(59)*x917 + x361*x921 + x420*x899 + x83*x889 + x891*x919 + x897*x922 + x923;
    x925 = parms(47)*x891 + x112*x890;
    x926 = x375 + x925;
    x927 = parms(41)*x907 + parms(42)*x478 + parms(43)*x910;
    x928 = parms(48)*x889 + x112*x473 + x176*x893 + x344*x914 + x369*x926 + x57*x912 + x61*x924 + x904*x916 + x927;
    x929 = x267 + x341;
    x930 = -x894;
    x931 = parms(53)*x908 + parms(55)*x909 + parms(56)*x910;
    x932 = parms(57)*x901 + x384*x906 + x439*x921 + x80*x917 + x895*x903 + x919*x930 + x931;
    x933 = parms(41)*x890 + parms(43)*x891 + x428;
    x934 = x425 + x933;
    x935 = x219*x891 + x433;
    x936 = x432 + x935;
    x937 = parms(43)*x907 + parms(45)*x478 + parms(46)*x910;
    x938 = parms(47)*x473 + x219*x900 + x351*x926 + x364*x934 + x431*x936 + x890*x916 + x932 + x937;
    x939 = parms(34) + x346;
    x940 = parms(31)*x176 + parms(35) + 2*x474 + x475;
    x941 = x176*x939 + x202*x929 + x349 + x46*x928 + x472 + x49*x938 + x940;
    x942 = -x890;
    x943 = parms(42)*x907 + parms(44)*x478 + parms(45)*x910;
    x944 = -parms(49)*x900 - x229*x889 - x352*x914 - x361*x936 - x57*x924 - x60*x912 - x891*x934 - x893*x942 - x943;
    x945 = parms(39) + x446;
    x946 = 2*parms(33)*x176 + parms(36)*x207 - x469 + x859;
    x947 = parms(38)*x344 + parms(39)*x202 + x207*x939 + x283*x344 + x443 + x444*x945 + x944 + x946;
    x948 = parms(59)*x909 + x80*x910;
    x949 = parms(60)*x917 + x894*x899 + x904*x906 + x948;
    x950 = parms(57)*x910 + x63*x908;
    x951 = parms(60)*x901 + x891*x921 + x899*x922 + x950;
    x952 = parms(47)*x910 + x112*x907;
    x953 = parms(38)*x37 + x136 + x445;
    x954 = -parms(50)*x473 + x457 - x57*x951 - x60*x949 - x891*x936 - x914*x942 - x952 + x953;
    x955 = parms(49)*x478 + x219*x910;
    x956 = parms(50)*x900 + x176*x914 + x57*x949 + x61*x951 + x904*x926 + x955;
    x957 = parms(58)*x908 + x83*x909;
    x958 = parms(48)*x907 + x229*x478;
    x959 = parms(50)*x889 + parms(60)*x889 + x364*x936 + x890*x926 + x895*x906 + x921*x930 + x957 + x958;
    x960 = parms(40)*x344 + x267 + x340 + x46*x956 + x462 + x49*x959;
    x961 = x156*x954 + x204*x960 + x31*x947 + x336 + x37*x941;
    x962 = parms(32)*x176 + parms(35)*x207;
    x963 = parms(37)*x473 + parms(39)*x344 + x339*x945 + x37*(parms(32) + x471) + x46*x938 + x473*x929 + x478*(parms(35) + x477) + x48*x928 + x962;
    x964 = x468 + x963;
    x965 = x31*x954 + x37*x960 + x483;
    x966 = parms(37)*x207 + x136*x176;
    x967 = x37*x945 + x46*x959 + x478*x929 + x48*x956 + x487 + x966;
    x968 = x9*x967;
    x969 = x176*x954 + x31*x960;
    x970 = x22*x969;
    x971 = x267 + x571;
    x972 = x49*x572;
    x973 = x580 + x892;
    x974 = x594 + x896;
    x975 = x596 + x898;
    x976 = x46*x572;
    x977 = x57*x649 + x61*x976;
    x978 = x599 + x902;
    x979 = x601 + x905;
    x980 = parms(58)*x972 + x585*x979 + x592*x975 + x63*x977 + x894*x974 + x904*x978 + x911;
    x981 = x583 + x913;
    x982 = x586 + x915;
    x983 = x57*x976 + x60*x649;
    x984 = x604 + x918;
    x985 = x606 + x920;
    x986 = parms(59)*x983 + x582*x985 + x608*x975 + x83*x972 + x891*x984 + x922*x974 + x923;
    x987 = x588 + x925;
    x988 = parms(48)*x972 + x112*x649 + x176*x973 + x57*x980 + x572*x981 + x585*x987 + x61*x986 + x904*x982 + x927;
    x989 = parms(34) + x573;
    x990 = parms(57)*x977 + x593*x979 + x619*x985 + x80*x983 + x895*x978 + x930*x984 + x931;
    x991 = x613 + x933;
    x992 = x616 + x935;
    x993 = parms(47)*x649 + x219*x976 + x364*x991 + x577*x987 + x615*x992 + x890*x982 + x937 + x990;
    x994 = a3*x971 + x176*x989 + x46*x988 + x49*x993 + x575 + x648 + x940;
    x995 = -parms(49)*x976 - x229*x972 - x57*x986 - x578*x981 - x582*x992 - x60*x980 - x891*x991 - x942*x973 - x943;
    x996 = parms(39) + x624;
    x997 = a3*parms(39) + parms(38)*x572 + x207*x989 + x283*x572 + x623 + x625*x996 + x946 + x995;
    x998 = parms(60)*x983 + x894*x975 + x904*x979 + x948;
    x999 = parms(60)*x977 + x891*x985 + x922*x975 + x950;
    x1000 = -parms(50)*x649 - x57*x999 - x60*x998 + x635 - x891*x992 - x942*x981 - x952 + x953;
    x1001 = parms(50)*x976 + x176*x981 + x57*x998 + x61*x999 + x904*x987 + x955;
    x1002 = parms(50)*x972 + parms(60)*x972 + x364*x992 + x890*x987 + x895*x979 + x930*x985 + x957 + x958;
    x1003 = parms(40)*x572 + x1001*x46 + x1002*x49 + x267 + x570 + x640;
    x1004 = parms(25) + x1000*x156 + x1003*x204 + x31*x997 + x37*x994;
    x1005 = parms(37)*x649 + parms(39)*x572 + x204*x996 + x37*(parms(32) + x647) + x46*x993 + x478*(parms(35) + x650) + x48*x988 + x649*x971 + x962;
    x1006 = x1005 + x646;
    x1007 = x1000*x31 + x1003*x37 + x654;
    x1008 = x1001*x48 + x1002*x46 + x293 + x37*x996 + x478*x971 + x966;
    x1009 = x1008*x9;
    x1010 = x1000*x176 + x1003*x31;
    x1011 = x1010*x22;
    x1012 = x33 - 1;
    x1013 = x1012*x229 + x745 + x95;
    x1014 = x769 + x93;
    x1015 = parms(45)*x1012 + x1014;
    x1016 = x51*x57;
    x1017 = x51*x61;
    x1018 = x1012*x60 + x67;
    x1019 = x1012*x57 + x76;
    x1020 = parms(58)*x1018 + x1019*x83 + x757;
    x1021 = parms(53)*x1018 + parms(55)*x1019 + x755 + x79;
    x1022 = x61*x744;
    x1023 = x1018*x63 + x52 + x765;
    x1024 = parms(52)*x1018 + parms(54)*x1019 + x762 + x88;
    x1025 = parms(51)*x1016 + parms(52)*x1017 + parms(53)*x139 + parms(58)*x800 + x1019*x1021 + x1020*x753 + x1022*x63 + x1023*x767 + x1024*x86;
    x1026 = x113 + x773;
    x1027 = x1026*x767;
    x1028 = x57*x744;
    x1029 = parms(59)*x1019 + x105 + x778;
    x1030 = parms(51)*x1018 + parms(52)*x1019 + x100 + x776;
    x1031 = -x1018;
    x1032 = parms(52)*x1016 + parms(54)*x1017 + parms(55)*x139 + parms(59)*x1028 + x1020*x781 + x1021*x1031 + x1029*x744 + x1030*x51 + x800*x83;
    x1033 = x110 + x771;
    x1034 = parms(44)*x1012 + x1033;
    x1035 = parms(41)*x51 + parms(43)*x139 + parms(48)*x800 + x1012*x1015 + x1013*x741 + x1025*x57 + x1027 + x1032*x61 + x1034*x86;
    x1036 = -x1019;
    x1037 = parms(53)*x1016 + parms(55)*x1017 + parms(56)*x139 + parms(57)*x1022 + x1018*x1024 + x1023*x754 + x1028*x80 + x1029*x788 + x1030*x1036;
    x1038 = x1026*x752;
    x1039 = parms(49)*x1012 + x128 + x790;
    x1040 = x125 + x793;
    x1041 = parms(42)*x1012 + x1040;
    x1042 = -x1012;
    x1043 = parms(46)*x139 + x1034*x66 + x1037 + x1038 + x1039*x792 + x1041*x1042 + x124 + x219*x744;
    x1044 = x119 + x784;
    x1045 = x134 + x796;
    x1046 = x1044*x17 + x1045*x33 + x786;
    x1047 = x1035*x46 + x1043*x49 + x1046 + x27*(x44 + x735);
    x1048 = -parms(42)*x51 - parms(45)*x139 - parms(49)*x744 - x1013*x800 - x1015*x139 - x1025*x60 - x1032*x57 - x1039*x744 - x1041*x51 - x229*x800;
    x1049 = x145 + x807;
    x1050 = x1045*x41 + x1049*x26 + x802;
    x1051 = x1048 + x1050 + x117*(x141 + x804);
    x1052 = parms(59)*x1017 + parms(60)*x1028 + x1019*x1020 + x1023*x86 + x139*x80;
    x1053 = parms(57)*x139 + parms(60)*x1022 + x1016*x63 + x1020*x1031 + x1029*x51;
    x1054 = x1049*x117 + x154;
    x1055 = -parms(47)*x139 - parms(49)*x86 - x1013*x139 - x1039*x51 - x1052*x60 - x1053*x57 + x1054;
    x1056 = x1026*x86;
    x1057 = x1012*x1013 + x1052*x57 + x1053*x61 + x1056 + x139*x219 + x745;
    x1058 = x1026*x66;
    x1059 = parms(48)*x51 + parms(50)*x800 + parms(58)*x1016 + parms(60)*x800 + x1017*x83 + x1018*x1023 + x1029*x1036 + x1039*x1042 + x1058;
    x1060 = x1044*x27 + x159;
    x1061 = x1057*x46 + x1059*x49 + x1060;
    x1062 = x1047*x37 + x1051*x31 + x1055*x156 + x1061*x204 + x817;
    x1063 = x1044*x759 + x1049*x740;
    x1064 = x1035*x48 + x1043*x46 + x1063 + x163*(x40 + x736) + x32*(x143 + x803);
    x1065 = x1064 + x821;
    x1066 = x1055*x31 + x1061*x37 + x169;
    x1067 = x1044*x163 + x1049*x32;
    x1068 = x1057*x48 + x1059*x46 + x1067 + x172;
    x1069 = x1068*x9;
    x1070 = x1055*x176 + x1061*x31 + x826;
    x1071 = x1070*x22;
    x1072 = -x57;
    x1073 = parms(53)*x61;
    x1074 = parms(55)*x1072 + x1073;
    x1075 = x1072*x1074;
    x1076 = -x61;
    x1077 = x1074*x1076;
    x1078 = -x1075*x60 - x1077*x57;
    x1079 = parms(45) + x1075*x57 + x1077*x61;
    x1080 = parms(52)*x61;
    x1081 = parms(54)*x1072;
    x1082 = x1080 + x1081;
    x1083 = parms(51)*x61;
    x1084 = parms(52)*x1072;
    x1085 = x1083 + x1084;
    x1086 = -x1072;
    x1087 = x1082*x61 + x1085*x1086;
    x1088 = -parms(42);
    x1089 = x1087 + x1088;
    x1090 = x1079*x46 + x1089*x49;
    x1091 = parms(58)*x61 + x1072*x83;
    x1092 = x1072*x1091;
    x1093 = x1076*x1091;
    x1094 = -x1092*x60 - x1093*x57;
    x1095 = x1092*x57 + x1093*x61 + x229;
    x1096 = ((x1072)*(x1072))*x63 + x112 + ((x61)*(x61))*x63;
    x1097 = x1095*x46 + x1096*x49;
    x1098 = x1078*x31 + x1090*x37 + x1094*x156 + x1097*x204;
    x1099 = x1079*x48 + x1089*x46;
    x1100 = x1095*x48 + x1096*x46;
    x1101 = x1100*x9;
    x1102 = x1094*x31 + x1097*x37;
    x1103 = x1094*x176 + x1097*x31;
    x1104 = x1103*x22;
    x1105 = x0*(x1098*x9 + x1099*x168 + x1101*x15 + x1102*x171 + x1104*x168) + x1*(d3*x1102*x9 + x1098*x11 + x1099*x9 + x1100*x171 + x1104*x9) - x1103*x6;
    x1106 = -x1105;
    x1107 = x176 - 1;
    x1108 = parms(45)*x1107 + x357;
    x1109 = x1108 + x354;
    x1110 = x1107*x57 + x381;
    x1111 = x1107*x60 + x387;
    x1112 = parms(53)*x1111 + parms(55)*x1110 + x390;
    x1113 = x1112 + x385;
    x1114 = parms(58)*x1111 + x1110*x83;
    x1115 = x1114 + x393;
    x1116 = x361*x61;
    x1117 = parms(52)*x1111 + parms(54)*x1110 + x399;
    x1118 = x1117 + x397;
    x1119 = x1111*x63 + x403;
    x1120 = x1119 + x402;
    x1121 = x356*x57;
    x1122 = x356*x61;
    x1123 = parms(51)*x1121 + parms(52)*x1122 + parms(53)*x448;
    x1124 = parms(58)*x352 + x1110*x1113 + x1115*x383 + x1116*x63 + x1118*x368 + x1120*x369 + x1123;
    x1125 = x1107*x229 + x363;
    x1126 = x1125 + x362;
    x1127 = x361*x57;
    x1128 = parms(51)*x1111 + parms(52)*x1110 + x411;
    x1129 = x1128 + x408;
    x1130 = parms(59)*x1110 + x416;
    x1131 = x1130 + x414;
    x1132 = -x1111;
    x1133 = parms(52)*x1121 + parms(54)*x1122 + parms(55)*x448;
    x1134 = parms(59)*x1127 + x1113*x1132 + x1115*x420 + x1129*x356 + x1131*x361 + x1133 + x352*x83;
    x1135 = parms(44)*x1107 + x371;
    x1136 = x1135 + x370;
    x1137 = parms(41)*x356 + parms(43)*x448;
    x1138 = x1107*x1109 + x1124*x57 + x1126*x344 + x1134*x61 + x1136*x368 + x1137 + x353 + x378;
    x1139 = -x1110;
    x1140 = parms(53)*x1121 + parms(55)*x1122 + parms(56)*x448;
    x1141 = parms(57)*x1116 + x1111*x1118 + x1120*x384 + x1127*x80 + x1129*x1139 + x1131*x439 + x1140;
    x1142 = parms(42)*x1107 + x427;
    x1143 = x1142 + x425;
    x1144 = -x1107;
    x1145 = parms(49)*x1107 + x434;
    x1146 = x1145 + x432;
    x1147 = parms(46)*x448 + x426;
    x1148 = parms(48)*x369 + x1136*x355 + x1141 + x1143*x1144 + x1146*x431 + x1147 + x424;
    x1149 = x1138*x46 + x1148*x49 + x350;
    x1150 = parms(42)*x356 + parms(45)*x448;
    x1151 = -parms(49)*x361 - x1109*x448 - x1124*x60 - x1126*x352 - x1134*x57 - x1143*x356 - x1146*x361 - x1150 - x229*x352;
    x1152 = x1151 + x447;
    x1153 = parms(59)*x1122 + x448*x80;
    x1154 = parms(60)*x1127 + x1110*x1115 + x1120*x368 + x1153;
    x1155 = parms(57)*x448 + x1121*x63;
    x1156 = parms(60)*x1116 + x1115*x1132 + x1131*x356 + x1155;
    x1157 = parms(47)*x448 + x112*x356;
    x1158 = -x1126*x448 - x1146*x356 - x1154*x60 - x1156*x57 - x1157 + x457;
    x1159 = x219*x448;
    x1160 = x1107*x1126 + x1154*x57 + x1156*x61 + x1159 + x362 + x459;
    x1161 = parms(58)*x1121 + x1122*x83;
    x1162 = parms(48)*x356;
    x1163 = parms(50)*x352 + parms(60)*x352 + x1111*x1120 + x1131*x1139 + x1144*x1146 + x1161 + x1162 + x463;
    x1164 = x1160*x46 + x1163*x49 + x462;
    x1165 = x1149*x37 + x1152*x31 + x1158*x156 + x1164*x204 + x336;
    x1166 = x1138*x48 + x1148*x46 + x479;
    x1167 = x1166 + x468;
    x1168 = x1158*x31 + x1164*x37 + x483;
    x1169 = x1160*x48 + x1163*x46 + x485 + x487;
    x1170 = x1169*x9;
    x1171 = x1158*x176 + x1164*x31;
    x1172 = x1171*x22;
    x1173 = x1108 + x580;
    x1174 = x1112 + x594;
    x1175 = x1114 + x596;
    x1176 = x582*x61;
    x1177 = x1117 + x599;
    x1178 = x1119 + x601;
    x1179 = parms(58)*x578 + x1110*x1174 + x1123 + x1175*x592 + x1176*x63 + x1177*x368 + x1178*x585;
    x1180 = x1125 + x583;
    x1181 = x57*x582;
    x1182 = x1128 + x604;
    x1183 = x1130 + x606;
    x1184 = parms(59)*x1181 + x1132*x1174 + x1133 + x1175*x608 + x1182*x356 + x1183*x582 + x578*x83;
    x1185 = x1135 + x586;
    x1186 = x1107*x1173 + x1137 + x1179*x57 + x1180*x572 + x1184*x61 + x1185*x368 + x579 + x590;
    x1187 = parms(57)*x1176 + x1111*x1177 + x1139*x1182 + x1140 + x1178*x593 + x1181*x80 + x1183*x619;
    x1188 = x1142 + x613;
    x1189 = x1145 + x616;
    x1190 = parms(48)*x585 + x1144*x1188 + x1147 + x1185*x355 + x1187 + x1189*x615 + x612;
    x1191 = x1186*x46 + x1190*x49 + x576;
    x1192 = -parms(49)*x582 - x1150 - x1173*x448 - x1179*x60 - x1180*x578 - x1184*x57 - x1188*x356 - x1189*x582 - x229*x578;
    x1193 = x1192 + x626;
    x1194 = parms(60)*x1181 + x1110*x1175 + x1153 + x1178*x368;
    x1195 = parms(60)*x1176 + x1132*x1175 + x1155 + x1183*x356;
    x1196 = -x1157 - x1180*x448 - x1189*x356 - x1194*x60 - x1195*x57 + x635;
    x1197 = x1107*x1180 + x1159 + x1194*x57 + x1195*x61 + x583 + x637;
    x1198 = parms(50)*x578 + parms(60)*x578 + x1111*x1178 + x1139*x1183 + x1144*x1189 + x1161 + x1162 + x641;
    x1199 = x1197*x46 + x1198*x49 + x640;
    x1200 = parms(25) + x1191*x37 + x1193*x31 + x1196*x156 + x1199*x204;
    x1201 = x1186*x48 + x1190*x46 + x651;
    x1202 = x1201 + x646;
    x1203 = x1196*x31 + x1199*x37 + x654;
    x1204 = x1197*x48 + x1198*x46 + x293 + x656;
    x1205 = x1204*x9;
    x1206 = x1196*x176 + x1199*x31;
    x1207 = x1206*x22;
    x1208 = x46*x57;
    x1209 = x46*x61;
    x1210 = x1072 + x829;
    x1211 = x61 + x830;
    x1212 = parms(53)*x1211 + parms(55)*x1210 + x832;
    x1213 = parms(52)*x1211 + parms(54)*x1210 + x835;
    x1214 = parms(51)*x1208 + parms(52)*x1209 + parms(53)*x49 + x1210*x1212 + x1213*x837;
    x1215 = parms(51)*x1211 + parms(52)*x1210 + x843;
    x1216 = -x1211;
    x1217 = parms(52)*x1208 + parms(54)*x1209 + parms(55)*x49 + x1212*x1216 + x1215*x46;
    x1218 = -parms(44) + x839;
    x1219 = parms(41)*x46 + 2*parms(43)*x49 + parms(45) + parms(46)*x837 + x1214*x57 + x1217*x61 + x1218*x837;
    x1220 = -x1210;
    x1221 = parms(53)*x1208 + parms(55)*x1209 + parms(56)*x49 + x1211*x1213 + x1215*x1220;
    x1222 = parms(46)*x49 + x1088 + x1218*x48 + x1221 + x854 + 2*x855;
    x1223 = parms(35) + x1219*x46 + x1222*x49;
    x1224 = -parms(42)*x46 - parms(45)*x49 - x1214*x60 - x1217*x57 - x46*(x1088 + x856) - x49*(-parms(45) + x853);
    x1225 = x1224 + x859;
    x1226 = parms(58)*x1211 + x1210*x83;
    x1227 = x1211*x63 + x863;
    x1228 = parms(59)*x1209 + x1210*x1226 + x1227*x837 + x49*x80;
    x1229 = parms(59)*x1210 + x868;
    x1230 = parms(57)*x49 + x1208*x63 + x1216*x1226 + x1229*x46;
    x1231 = -parms(47)*x49 - x112*x46 - x1228*x60 - x1230*x57 + x136 - x46*(parms(48)*x837 + x112) - x49*(parms(47) + parms(48)*x48);
    x1232 = parms(48)*x49 + x1228*x57 + x1230*x61 + x219*x49 + x229 + x875;
    x1233 = parms(58)*x1208 + x112 + x1209*x83 + x1211*x1227 + x1220*x1229 + x877;
    x1234 = x1232*x46 + x1233*x49 + x267;
    x1235 = x1223*x37 + x1225*x31 + x1231*x156 + x1234*x204;
    x1236 = x1219*x48 + x1222*x46;
    x1237 = x1232*x48 + x1233*x46;
    x1238 = x1237*x9;
    x1239 = x1231*x31 + x1234*x37;
    x1240 = x1231*x176 + x1234*x31;
    x1241 = x1240*x22;
    x1242 = x40 + x43 + x735;
    x1243 = x745 + x98;
    x1244 = x757 + x84;
    x1245 = x51 + 1;
    x1246 = parms(56)*x1245 + x755 + x78;
    x1247 = parms(57)*x1245 + x70 + x765;
    x1248 = parms(55)*x1245 + x762 + x87;
    x1249 = -x1245;
    x1250 = parms(51)*x77 + parms(52)*x107 + x1244*x753 + x1246*x77 + x1247*x767 + x1248*x1249 + x63*x781;
    x1251 = x1014 + x91;
    x1252 = x104 + x1245*x80 + x778;
    x1253 = parms(53)*x1245 + x102 + x776;
    x1254 = parms(54)*x107 + parms(59)*x753 + x101 + x107*x1246 + x1244*x781 + x1245*x1253 + x1252*x744;
    x1255 = x1033 + x109;
    x1256 = x1027 + x1243*x741 + x1250*x57 + x1251*x33 + x1254*x61 + x1255*x86;
    x1257 = parms(53)*x77 + parms(55)*x107 + parms(57)*x781 + x121*x1253 + x1247*x754 + x1248*x69 + x1252*x788 + x753*x80;
    x1258 = x129 + x790;
    x1259 = x1040 + x123;
    x1260 = x1038 + x1255*x66 + x1257 + x1258*x792 + x1259*x96;
    x1261 = x1046 + x1242*x27 + x1256*x46 + x1260*x49;
    x1262 = -x1243*x800 - x1250*x60 - x1251*x139 - x1254*x57 - x1258*x744 - x1259*x51;
    x1263 = x141 + x142 + x803;
    x1264 = x1050 + x117*x1263 + x1262;
    x1265 = parms(59)*x107 + x1244*x77 + x1247*x1249 + x765;
    x1266 = parms(60)*x781 + x107*x1244 + x1245*x1252 + x63*x77;
    x1267 = x1054 - x1243*x139 - x1258*x51 - x1265*x60 - x1266*x57;
    x1268 = x1056 + x1243*x33 + x1265*x57 + x1266*x61;
    x1269 = parms(58)*x77 + x1058 + x107*x83 + x121*x1252 + x1247*x69 + x1258*x96;
    x1270 = x1060 + x1268*x46 + x1269*x49;
    x1271 = x1261*x37 + x1264*x31 + x1267*x156 + x1270*x204 + x817;
    x1272 = x1063 + x1242*x163 + x1256*x48 + x1260*x46 + x1263*x32;
    x1273 = x1272 + x821;
    x1274 = x1267*x31 + x1270*x37 + x169;
    x1275 = x1067 + x1268*x48 + x1269*x46 + x172;
    x1276 = x1275*x9;
    x1277 = x1267*x176 + x1270*x31 + x826;
    x1278 = x1277*x22;
    x1279 = -parms(55);
    x1280 = -parms(53)*x57 - x1279*x60;
    x1281 = x1073 + x1279*x57;
    x1282 = x1281*x46;
    x1283 = -x57*x80 - x60*x83;
    x1284 = x57*x83 + x61*x80;
    x1285 = x1284*x46;
    x1286 = x1280*x31 + x1282*x37 + x1283*x156 + x1285*x204;
    x1287 = x1281*x48;
    x1288 = x1284*x48;
    x1289 = x1288*x9;
    x1290 = x1283*x31 + x1285*x37;
    x1291 = x1283*x176 + x1285*x31;
    x1292 = x1291*x22;
    x1293 = x0*(x1286*x9 + x1287*x168 + x1289*x15 + x1290*x171 + x1292*x168) + x1*(d3*x1290*x9 + x11*x1286 + x1287*x9 + x1288*x171 + x1292*x9) - x1291*x6;
    x1294 = -x1293;
    x1295 = x356 + 1;
    x1296 = parms(56)*x1295 + x389;
    x1297 = x1296 + x385;
    x1298 = parms(55)*x1295 + x398;
    x1299 = x1298 + x397;
    x1300 = -x1295;
    x1301 = parms(57)*x1295 + x404;
    x1302 = x1301 + x402;
    x1303 = parms(51)*x382 + parms(52)*x419;
    x1304 = x1297*x382 + x1299*x1300 + x1302*x369 + x1303 + x396 + x420*x63;
    x1305 = parms(53)*x1295 + x410;
    x1306 = x1305 + x408;
    x1307 = x1295*x80 + x415;
    x1308 = x1307 + x414;
    x1309 = parms(54)*x419 + x409;
    x1310 = parms(59)*x383 + x1295*x1306 + x1297*x419 + x1308*x361 + x1309 + x421;
    x1311 = x1304*x57 + x1310*x61 + x379;
    x1312 = parms(53)*x382 + parms(55)*x419;
    x1313 = parms(57)*x420 + x1299*x388 + x1302*x384 + x1306*x438 + x1308*x439 + x1312 + x383*x80;
    x1314 = x1313 + x437;
    x1315 = x1311*x46 + x1314*x49 + x350;
    x1316 = -x1304*x60 - x1310*x57 - x449;
    x1317 = x1316 + x447;
    x1318 = parms(59)*x419;
    x1319 = x1300*x1302 + x1318 + x402 + x453;
    x1320 = x382*x63;
    x1321 = parms(60)*x420 + x1295*x1308 + x1320 + x455;
    x1322 = -x1319*x60 - x1321*x57 - x452 + x457;
    x1323 = x1319*x57 + x1321*x61 + x460;
    x1324 = parms(58)*x382 + x419*x83;
    x1325 = x1302*x388 + x1308*x438 + x1324 + x464;
    x1326 = x1323*x46 + x1325*x49 + x462;
    x1327 = x1315*x37 + x1317*x31 + x1322*x156 + x1326*x204 + x336;
    x1328 = x1311*x48 + x1314*x46 + x479;
    x1329 = x1328 + x468;
    x1330 = x1322*x31 + x1326*x37 + x483;
    x1331 = x1323*x48 + x1325*x46 + x485 + x487;
    x1332 = x1331*x9;
    x1333 = x1322*x176 + x1326*x31;
    x1334 = x1333*x22;
    x1335 = x1296 + x594;
    x1336 = x1298 + x599;
    x1337 = x1301 + x601;
    x1338 = x1300*x1336 + x1303 + x1335*x382 + x1337*x585 + x598 + x608*x63;
    x1339 = x1305 + x604;
    x1340 = x1307 + x606;
    x1341 = parms(59)*x592 + x1295*x1339 + x1309 + x1335*x419 + x1340*x582 + x609;
    x1342 = x1338*x57 + x1341*x61 + x591;
    x1343 = parms(57)*x608 + x1312 + x1336*x388 + x1337*x593 + x1339*x438 + x1340*x619 + x592*x80;
    x1344 = x1343 + x618;
    x1345 = x1342*x46 + x1344*x49 + x576;
    x1346 = -x1338*x60 - x1341*x57 - x627;
    x1347 = x1346 + x626;
    x1348 = x1300*x1337 + x1318 + x601 + x631;
    x1349 = parms(60)*x608 + x1295*x1340 + x1320 + x633;
    x1350 = -x1348*x60 - x1349*x57 - x630 + x635;
    x1351 = x1348*x57 + x1349*x61 + x638;
    x1352 = x1324 + x1337*x388 + x1340*x438 + x642;
    x1353 = x1351*x46 + x1352*x49 + x640;
    x1354 = parms(25) + x1345*x37 + x1347*x31 + x1350*x156 + x1353*x204;
    x1355 = x1342*x48 + x1344*x46 + x651;
    x1356 = x1355 + x646;
    x1357 = x1350*x31 + x1353*x37 + x654;
    x1358 = x1351*x48 + x1352*x46 + x293 + x656;
    x1359 = x1358*x9;
    x1360 = x1350*x176 + x1353*x31;
    x1361 = x1360*x22;
    x1362 = x46 + 1;
    x1363 = parms(56)*x1362 + x831;
    x1364 = parms(55)*x1362 + x834;
    x1365 = -x1362;
    x1366 = parms(51)*x829 + parms(52)*x845 + x1363*x829 + x1364*x1365;
    x1367 = parms(53)*x1362 + x842;
    x1368 = parms(54)*x845 + x1362*x1367 + x1363*x845 + x841;
    x1369 = x1366*x57 + x1368*x61 + x840;
    x1370 = parms(53)*x829 + parms(55)*x845 + x1364*x830 + x1367*x849;
    x1371 = x1370 + x848;
    x1372 = parms(35) + x1369*x46 + x1371*x49;
    x1373 = -x1366*x60 - x1368*x57 - x857;
    x1374 = x1373 + x859;
    x1375 = parms(57)*x1362 + x864;
    x1376 = parms(59)*x845 + x1365*x1375 + x862;
    x1377 = x1362*x80 + x867;
    x1378 = x1362*x1377 + x63*x829 + x870;
    x1379 = x136 - x1376*x60 - x1378*x57 - x872;
    x1380 = x1376*x57 + x1378*x61 + x875;
    x1381 = parms(58)*x829 + x1375*x830 + x1377*x849 + x83*x845 + x877;
    x1382 = x1380*x46 + x1381*x49 + x267;
    x1383 = x1372*x37 + x1374*x31 + x1379*x156 + x1382*x204;
    x1384 = x1369*x48 + x1371*x46;
    x1385 = x1380*x48 + x1381*x46;
    x1386 = x1385*x9;
    x1387 = x1379*x31 + x1382*x37;
    x1388 = x1379*x176 + x1382*x31;
    x1389 = x1388*x22;
    x1390 = parms(56) + x1074;
    x1391 = parms(51)*x1072 + parms(52)*x1076 + x1072*x1390 - x1080 - x1081 + x1279;
    x1392 = parms(53) + parms(54)*x1076 + x1076*x1390 + x1083 + 2*x1084;
    x1393 = -x1391*x60 - x1392*x57;
    x1394 = parms(45) + x1391*x57 + x1392*x61;
    x1395 = parms(53)*x1072 + parms(55)*x1076 + x1086*(parms(53) + x1085) + x61*(parms(55) + x1082);
    x1396 = x1088 + x1395;
    x1397 = x1394*x46 + x1396*x49;
    x1398 = parms(59)*x1076 + parms(59)*x61 + x1092 + x83;
    x1399 = x1093 + x80;
    x1400 = -x1398*x60 - x1399*x57;
    x1401 = x1398*x57 + x1399*x61 + x229;
    x1402 = parms(58)*x1072 + x1076*x83 + x1086*(parms(59)*x1072 + x80) + x112 + x61*(parms(57) + x61*x63);
    x1403 = x1401*x46 + x1402*x49;
    x1404 = x1393*x31 + x1397*x37 + x1400*x156 + x1403*x204;
    x1405 = x1394*x48 + x1396*x46;
    x1406 = x1401*x48 + x1402*x46;
    x1407 = x1406*x9;
    x1408 = x1400*x31 + x1403*x37;
    x1409 = x1400*x176 + x1403*x31;
    x1410 = x1409*x22;
    x1411 = parms(17)*x20 + x306 + x307;
    x1412 = x331 + x332;
    x1413 = x0*x1411 + x1412*x184;
    x1414 = x27*(parms(28)*x17 + x312);
    x1415 = parms(26)*x27 + parms(27)*x25 + x303;
    x1416 = -x36;
    x1417 = -x138*x31 - x1414 - x1416*x19 - x148*x176 - x155*x161 - x156*x160 - x166*x17 - x28*(parms(28)*x1416 + x1415);
    x1418 = x179*x185;
    x1419 = a2*(x11*x170 + x1418 + x174) + x1413 + x1417 + x173*x22;
    x1420 = -parms(25) + x1415;
    x1421 = -parms(22)*x188 - parms(25)*x191 - parms(29)*x199 - x156*x302 - x161*x299 - x176*x289 + x194*x292 - x196*x294 - x203*x318 - x27*x315 - x28*(x1420 - x195) - x280*x31;
    x1422 = -x1419;
    x1423 = x202*x487 + x663*(parms(27) + x482);
    x1424 = -x1423 - x156*x466 - x161*x458 - x176*x451 - x31*x442;
    x1425 = a2*parms(18);
    x1426 = a2*(x11*x484 + x328 + x489) + x1424 + x1425 + x22*x488;
    x1427 = -x1426;
    x1428 = x192*x316;
    x1429 = -parms(22)*x27 - parms(25)*x28 - parms(29)*x17 - x156*x557 - x161*x554 - x176*x547 - x27*(x314 + x560) - x28*(x1420 + x1428) - x294*x494 - x31*x542 - x494*x549 - x499*x563;
    x1430 = a3*x293;
    x1431 = -x1430 - x156*x644 - x161*x636 - x176*x629 - x31*x622;
    x1432 = a2*(x11*x655 + x658) + x1431 + x22*x657;
    x1433 = -x1432;
    x1434 = -parms(29)*x664 - x156*x722 - x161*x719 - x176*x716 - x294*x663 - x31*x712 - x663*(2*parms(27) + x727) - x666*(-2*parms(29) + x486);
    x1435 = x1414 + x17*x820 + x19*x494 + x28*(x1415 + x1428);
    x1436 = -x1435 - x156*x815 - x161*x812 - x176*x809 - x31*x798;
    x1437 = -x156*x879 - x161*x873 - x176*x860 - x31*x852;
    x1438 = a2*(x11*x884 + x883) + x1437 + x22*x882;
    x1439 = -x1438;
    x1440 = -x1423 - x156*x960 - x161*x954 - x176*x947 - x31*x941;
    x1441 = -x1000*x161 - x1003*x156 - x1430 - x176*x997 - x31*x994;
    x1442 = -x1047*x31 - x1051*x176 - x1055*x161 - x1061*x156 - x1435;
    x1443 = -x1078*x176 - x1090*x31 - x1094*x161 - x1097*x156;
    x1444 = a2*(x11*x1102 + x1101) + x1100*x22 + x1443;
    x1445 = -x1444;
    x1446 = -x1149*x31 - x1152*x176 - x1158*x161 - x1164*x156 - x1423;
    x1447 = -x1191*x31 - x1193*x176 - x1196*x161 - x1199*x156 - x1430;
    x1448 = -x1223*x31 - x1225*x176 - x1231*x161 - x1234*x156;
    x1449 = -x1261*x31 - x1264*x176 - x1267*x161 - x1270*x156 - x1435;
    x1450 = -x1280*x176 - x1282*x31 - x1283*x161 - x1285*x156;
    x1451 = a2*(x11*x1290 + x1289) + x1288*x22 + x1450;
    x1452 = -x1451;
    x1453 = -x1315*x31 - x1317*x176 - x1322*x161 - x1326*x156 - x1423;
    x1454 = -x1345*x31 - x1347*x176 - x1350*x161 - x1353*x156 - x1430;
    x1455 = -x1372*x31 - x1374*x176 - x1379*x161 - x1382*x156;
    x1456 = -x1393*x176 - x1397*x31 - x1400*x161 - x1403*x156;
    x1457 = a3*x173 + x1417;
    x1458 = -x1457;
    x1459 = a3*x488 + x1424;
    x1460 = -x1459;
    x1461 = a3*x657 + x1431;
    x1462 = -x1461;
    x1463 = a3*x882 + x1437;
    x1464 = -x1463;
    x1465 = a3*x1100 + x1443;
    x1466 = -x1465;
    x1467 = a3*x1288 + x1450;
    x1468 = -x1467;
    x1469 = -x164;
    x1470 = -x480;
    x1471 = -x652;
    x1472 = -x881;
    x1473 = -x1099;
    x1474 = -x1287;
    x1475 = -x140;
    x1476 = -x450;
    x1477 = -x628;
    x1478 = -x858;
    x1479 = -x1078;
    x1480 = -x1280;
    x1481 = -x122;
    x1482 = -x440;
    x1483 = -x620;
    x1484 = -x850;
    x1485 = -x1087;

    C = zeros(36,1);
    
    C(1) = dq(1)*x183;
    C(2) = dq(1)*(x0*(a2*x185 + parms(11)*x1 + parms(12)*x179 + parms(17)*x6 + parms(18)*x186 + x1*x187 + x15*x324 + x168*x319 + x168*x326 + x171*x322 + x20*x320 + x305*x9 - x306 - x307 + x327) + x1*(d3*x322*x9 + parms(14)*x179 + x11*x305 + x171*x323 + x179*x187 + x186*x330 + x319*x9 + x326*x9 + x329*x6 + 2*x331 + x332 + x333) + x334 + x493 + x6*(parms(18)*x1 + parms(20)*x186 + x0*x320 + x179*x330 + x184*x329 - x325)) + dq(2)*x492;
    C(3) = dq(1)*(x0*(x15*x567 + x168*x564 + x168*x569 + x171*x565 + x558*x9 + x8) + x1*(d3*x565*x9 + x11*x558 + x171*x566 + x180 + x564*x9 + x569*x9) + x334 + x6*(x182 - x568) + x662) + dq(2)*(x0*(x15*x730 + x168*x726 + x168*x732 + x171*x728 + x327 + x723*x9) + x1*(d3*x728*x9 + x11*x723 + x171*x729 + x333 + x726*x9 + x732*x9) + x493 - x6*x731 + x662) + dq(3)*x661;
    C(4) = dq(1)*(x0*(x15*x825 + x168*x822 + x168*x828 + x171*x823 + x8 + x818*x9) + x1*(d3*x823*x9 + x11*x818 + x171*x824 + x180 + x822*x9 + x828*x9) + x334 + x6*(x182 - x827) + x888) + dq(2)*(x0*(x15*x968 + x168*x964 + x168*x970 + x171*x965 + x327 + x9*x961) + x1*(d3*x9*x965 + x11*x961 + x171*x967 + x333 + x9*x964 + x9*x970) + x493 - x6*x969 + x888) + dq(3)*(x0*(x1004*x9 + x1006*x168 + x1007*x171 + x1009*x15 + x1011*x168) + x1*(d3*x1007*x9 + x1004*x11 + x1006*x9 + x1008*x171 + x1011*x9) - x1010*x6 + x662 + x888) + dq(4)*x887;
    C(5) = dq(1)*(x0*(x1062*x9 + x1065*x168 + x1066*x171 + x1069*x15 + x1071*x168 + x8) + x1*(d3*x1066*x9 + x1062*x11 + x1065*x9 + x1068*x171 + x1071*x9 + x180) + x1106 + x334 + x6*(-x1070 + x182)) + dq(2)*(x0*(x1165*x9 + x1167*x168 + x1168*x171 + x1170*x15 + x1172*x168 + x327) + x1*(d3*x1168*x9 + x11*x1165 + x1167*x9 + x1169*x171 + x1172*x9 + x333) + x1106 - x1171*x6 + x493) + dq(3)*(x0*(x1200*x9 + x1202*x168 + x1203*x171 + x1205*x15 + x1207*x168) + x1*(d3*x1203*x9 + x11*x1200 + x1202*x9 + x1204*x171 + x1207*x9) + x1106 - x1206*x6 + x662) + dq(4)*(x0*(x1235*x9 + x1236*x168 + x1238*x15 + x1239*x171 + x1241*x168) + x1*(d3*x1239*x9 + x11*x1235 + x1236*x9 + x1237*x171 + x1241*x9) + x1106 - x1240*x6 + x888) + dq(5)*x1105;
    C(6) = dq(1)*(x0*(x1271*x9 + x1273*x168 + x1274*x171 + x1276*x15 + x1278*x168 + x8) + x1*(d3*x1274*x9 + x11*x1271 + x1273*x9 + x1275*x171 + x1278*x9 + x180) + x1294 + x334 + x6*(-x1277 + x182)) + dq(2)*(x0*(x1327*x9 + x1329*x168 + x1330*x171 + x1332*x15 + x1334*x168 + x327) + x1*(d3*x1330*x9 + x11*x1327 + x1329*x9 + x1331*x171 + x1334*x9 + x333) + x1294 - x1333*x6 + x493) + dq(3)*(x0*(x1354*x9 + x1356*x168 + x1357*x171 + x1359*x15 + x1361*x168) + x1*(d3*x1357*x9 + x11*x1354 + x1356*x9 + x1358*x171 + x1361*x9) + x1294 - x1360*x6 + x662) + dq(4)*(x0*(x1383*x9 + x1384*x168 + x1386*x15 + x1387*x171 + x1389*x168) + x1*(d3*x1387*x9 + x11*x1383 + x1384*x9 + x1385*x171 + x1389*x9) + x1294 - x1388*x6 + x888) + dq(5)*(x0*(x1404*x9 + x1405*x168 + x1407*x15 + x1408*x171 + x1410*x168) + x1*(d3*x1408*x9 + x11*x1404 + x1405*x9 + x1406*x171 + x1410*x9) + x1106 + x1294 - x1409*x6) + dq(6)*x1293;
    C(7) = dq(1)*x1419;
    C(8) = dq(1)*(a2*(x11*x322 + x1418 + x324 + x328) + parms(13)*x1 + parms(15)*x179 + x0*(parms(15) + x1411) + x1421 + x1422 + x1427 + x184*(x1412 + x333) + x22*x323 + x329*x4) + dq(2)*x1426;
    C(9) = dq(1)*(a2*(x11*x565 + x1418 + x567) + x1413 + x1422 + x1429 + x1433 + x22*x566) + dq(2)*(a2*(x11*x728 + x328 + x730) + x1425 + x1427 + x1433 + x1434 + x22*x729) + dq(3)*x1432;
    C(10) = dq(1)*(a2*(x11*x823 + x1418 + x825) + x1413 + x1422 + x1436 + x1439 + x22*x824) + dq(2)*(a2*(x11*x965 + x328 + x968) + x1425 + x1427 + x1439 + x1440 + x22*x967) + dq(3)*(a2*(x1007*x11 + x1009) + x1008*x22 + x1433 + x1439 + x1441) + dq(4)*x1438;
    C(11) = dq(1)*(a2*(x1066*x11 + x1069 + x1418) + x1068*x22 + x1413 + x1422 + x1442 + x1445) + dq(2)*(a2*(x11*x1168 + x1170 + x328) + x1169*x22 + x1425 + x1427 + x1445 + x1446) + dq(3)*(a2*(x11*x1203 + x1205) + x1204*x22 + x1433 + x1445 + x1447) + dq(4)*(a2*(x11*x1239 + x1238) + x1237*x22 + x1439 + x1445 + x1448) + dq(5)*x1444;
    C(12) = dq(1)*(a2*(x11*x1274 + x1276 + x1418) + x1275*x22 + x1413 + x1422 + x1449 + x1452) + dq(2)*(a2*(x11*x1330 + x1332 + x328) + x1331*x22 + x1425 + x1427 + x1452 + x1453) + dq(3)*(a2*(x11*x1357 + x1359) + x1358*x22 + x1433 + x1452 + x1454) + dq(4)*(a2*(x11*x1387 + x1386) + x1385*x22 + x1439 + x1452 + x1455) + dq(5)*(a2*(x11*x1408 + x1407) + x1406*x22 + x1445 + x1452 + x1456) + dq(6)*x1451;
    C(13) = dq(1)*x1457;
    C(14) = dq(1)*(a3*x323 + x1421 + x1458 + x1460) + dq(2)*x1459;
    C(15) = dq(1)*(a3*x566 + x1429 + x1458 + x1462) + dq(2)*(a3*x729 + x1434 + x1460 + x1462) + dq(3)*x1461;
    C(16) = dq(1)*(a3*x824 + x1436 + x1458 + x1464) + dq(2)*(a3*x967 + x1440 + x1460 + x1464) + dq(3)*(a3*x1008 + x1441 + x1462 + x1464) + dq(4)*x1463;
    C(17) = dq(1)*(a3*x1068 + x1442 + x1458 + x1466) + dq(2)*(a3*x1169 + x1446 + x1460 + x1466) + dq(3)*(a3*x1204 + x1447 + x1462 + x1466) + dq(4)*(a3*x1237 + x1448 + x1464 + x1466) + dq(5)*x1465;
    C(18) = dq(1)*(a3*x1275 + x1449 + x1458 + x1468) + dq(2)*(a3*x1331 + x1453 + x1460 + x1468) + dq(3)*(a3*x1358 + x1454 + x1462 + x1468) + dq(4)*(a3*x1385 + x1455 + x1464 + x1468) + dq(5)*(a3*x1406 + x1456 + x1466 + x1468) + dq(6)*x1467;
    C(19) = dq(1)*x164;
    C(20) = dq(1)*(x1469 + x1470 + x309) + dq(2)*x480;
    C(21) = dq(1)*(x1469 + x1471 + x559) + dq(2)*(x1470 + x1471 + x725) + dq(3)*x652;
    C(22) = dq(1)*(x1469 + x1472 + x819) + dq(2)*(x1470 + x1472 + x963) + dq(3)*(x1005 + x1471 + x1472) + dq(4)*x881;
    C(23) = dq(1)*(x1064 + x1469 + x1473) + dq(2)*(x1166 + x1470 + x1473) + dq(3)*(x1201 + x1471 + x1473) + dq(4)*(x1236 + x1472 + x1473) + dq(5)*x1099;
    C(24) = dq(1)*(x1272 + x1469 + x1474) + dq(2)*(x1328 + x1470 + x1474) + dq(3)*(x1355 + x1471 + x1474) + dq(4)*(x1384 + x1472 + x1474) + dq(5)*(x1405 + x1473 + x1474) + dq(6)*x1287;
    C(25) = dq(1)*x140;
    C(26) = dq(1)*(x1475 + x1476 + x282) + dq(2)*x450;
    C(27) = dq(1)*(x1475 + x1477 + x543) + dq(2)*(x1476 + x1477 + x714) + dq(3)*x628;
    C(28) = dq(1)*(x1475 + x1478 + x801) + dq(2)*(x1476 + x1478 + x944) + dq(3)*(x1477 + x1478 + x995) + dq(4)*x858;
    C(29) = dq(1)*(x1048 + x1475 + x1479) + dq(2)*(x1151 + x1476 + x1479) + dq(3)*(x1192 + x1477 + x1479) + dq(4)*(x1224 + x1478 + x1479) + dq(5)*x1078;
    C(30) = dq(1)*(x1262 + x1475 + x1480) + dq(2)*(x1316 + x1476 + x1480) + dq(3)*(x1346 + x1477 + x1480) + dq(4)*(x1373 + x1478 + x1480) + dq(5)*(x1393 + x1479 + x1480) + dq(6)*x1280;
    C(31) = dq(1)*x122;
    C(32) = dq(1)*(x1481 + x1482 + x273) + dq(2)*x440;
    C(33) = dq(1)*(x1481 + x1483 + x538) + dq(2)*(x1482 + x1483 + x707) + dq(3)*x620;
    C(34) = dq(1)*(x1481 + x1484 + x789) + dq(2)*(x1482 + x1484 + x932) + dq(3)*(x1483 + x1484 + x990) + dq(4)*x850;
    C(35) = dq(1)*(x1037 + x1481 + x1485) + dq(2)*(x1141 + x1482 + x1485) + dq(3)*(x1187 + x1483 + x1485) + dq(4)*(x1221 + x1484 + x1485) + dq(5)*x1087;
    C(36) = dq(1)*(x1257 + x1481) + dq(2)*(x1313 + x1482) + dq(3)*(x1343 + x1483) + dq(4)*(x1370 + x1484) + dq(5)*(x1395 + x1485);


    C_out = reshape(C,6,6)';

end
